simulink model "MotorXploer"  (R2024b)
settings: Solver=FixedStepAuto  StartTime=0.0  StopTime=inf  FixedStep=0.001  RelTol=1e-3  EnableMultiTasking=on
values from neighbouring files (symbols this model uses):
  n = (-(230/0.2)*((Torque1).^2) + 230*Torque1) ./ (((5-0.98)/0.2)*Torque1*12 + 0.98*12)*100    [UnitedPlot.m]
undefined symbols (not defined in the file or in its folder): Blocking, LF, Non
libraries: hdlsllib x5, amg_usbconverter_n_connect_lib x3, cstblocks x1, simulink x1, waijung_addon_module x1
(part 1 of 2)
settings Model: Creator=beamk  LastModifiedBy=KATANA
settings OptimizationCC: DefaultParameterBehavior=Inlined  EnhancedBackFolding=on  PassReuseOutputArgsAs=Individual arguments  ZeroExternalMemoryAtStartup=off  ZeroInternalMemoryAtStartup=off  MaxStackSize=64  OptimizeBlockOrder=speed  DifferentSizesBufferReuse=on  OptimizationCustomize=off  EfficientTunableParamExpr=on
settings DebuggingCC: ParameterTunabilityLossMsg=error
settings HardwareCC: ProdBitPerPointer=32  ProdBitPerSizeT=32  ProdBitPerPtrDiffT=32  ProdLargestAtomicInteger=Long  ProdLargestAtomicFloat=Double  ProdWordSize=32  ProdLongLongMode=on  ProdHWDeviceType=ARM Compatible->ARM Cortex-M
settings SFSimCC: MATLABDynamicMemAlloc=off
settings RTWCC: Description=Embedded Coder  SystemTargetFile=ert.tlc  HardwareBoard=STM32G4xx Based  TemplateMakefile=ert_default_tmf  Toolchain=GNU Tools for ARM Embedded Processors
settings CodeAppCC: ForceParamTrailComments=on  IgnoreCustomStorageClasses=off  OperatorAnnotations=on  SimulinkDataObjDesc=on  SFDataObjDesc=on  InsertBlockDesc=on
settings ERTTargetCC: TargetLangStandard=C99 (ISO)  CodeReplacementLibrary=ARM Cortex-M  ExtModeTransport=3  ExtModeStaticAlloc=on  ExtModeStaticAllocSize=2048  ExtModeMexFile=ext_xcp  ExtModeIntrfLevel=Level2 - Open

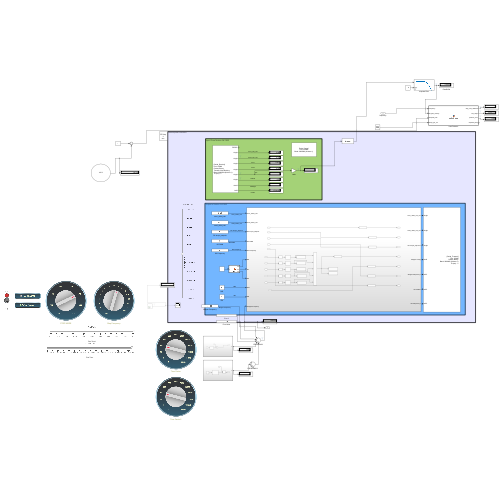
[thumbnail: Simulink's stored preview of the top-level diagram]
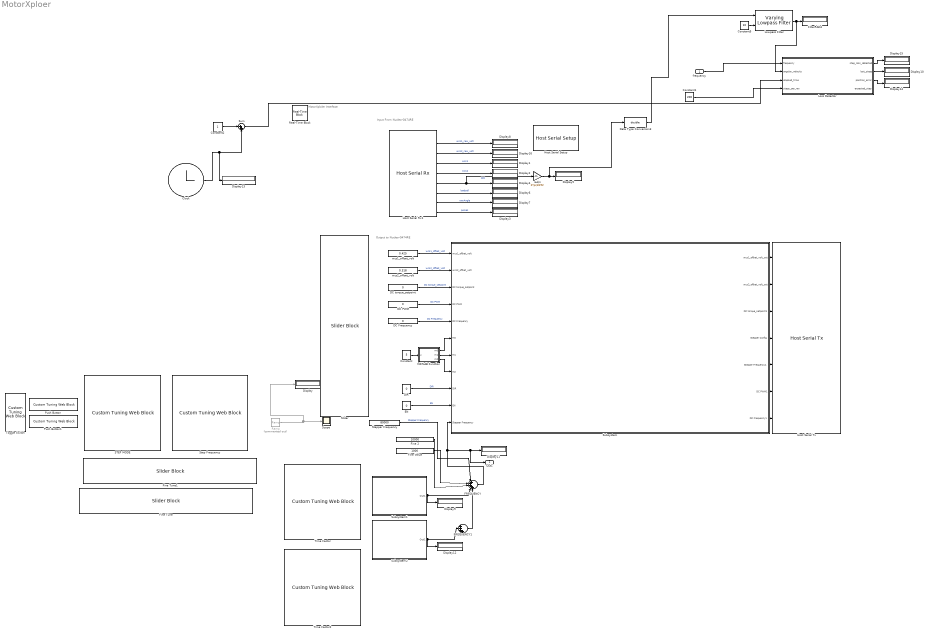
== system MotorXploer ==
  note: Output to Nucleo-G474RE
  note: Input From Nucleo-G474RE
  note: MotorXploler Interface
  frequency : Inport
  Clock : Clock
  Constant : Constant  Value=5
  Constant1 : Constant  Value=200
  Constant2 : Constant
  Constant5 : Constant  Value=10
  DC Frequency : Constant  Value=0
  DC PWM : Constant  Value=0
  DC torque_setpoint : Constant  Value=0
  DIR : Constant  Value=0  OutDataTypeStr=uint8
  Data Type Conversion3 : DataTypeConversion  OutDataTypeStr=double  SaturateOnIntegerOverflow=off  RndMeth=Floor
  Display{,1..16} (17 alike) : Display
  EN : Constant  Value=0  OutDataTypeStr=uint8
  FREQUENCY : Sum  Inputs=|+++++
  FREQUENCY1 : Sum  Inputs=|++++
  FilterRAD4 : Display
  Fine 2 : Constant  Value=10000
  Fine Tune : SliderBlock  ScaleMax=1000
  Fine Tune1 : SliderBlock  ScaleMax=10000  TickInterval=1000
  Fine Value : Constant  Value=1000
  Host Serial Rx1 : amg_usbconverter_n_connect_lib/Host Serial Rx  conf=rx  port=<auto>  baudrate=2000000  databits=8  parity=None  stopbit=1  flowcontrol=None  transfer=Non-Blocking  timeout=5  packetmode=Binary  enableinitialvalues=off  initialvalues=[]  binheader='45'  binterminator='A'  porttype_double=0  porttype_single=6  porttype_int8=0  porttype_uint8=0  porttype_int16=0  porttype_uint16=1  porttype_int32=1  porttype_uint32=0  asciiformat='%f,%f,%d,%d'  rx_asciiterminator="LF (0x0A - \"\\n\")"  tx_asciiterminator="CRLF (0x0D 0x0A - \"\\r\\n\")"  sampletime=-1  enablecustomportlabel=off  cinputportlabel=0  coutputportlabel=A  portpinstr=0  blockid=HostSerialRx1  inputporttype=[]  inputportwidth=[]  inputportlabel={}  outputporttype=[3 1 1 1 1 1 1 5 6]  outputportwidth=[1 1 1 1 1 1 1 1 1]  outputportlabel={'READY','single','single','single','single','single','single','uint16','int32'}  compat=0  optionstring=[]  autoport='COM17'
  Host Serial Setup : amg_usbconverter_n_connect_lib/Host Serial Setup  conf=setup  port=<auto>  baudrate=2000000  databits=8  parity=None  stopbit=1  flowcontrol=None  transfer=Blocking  timeout=2  packetmode=Binary  initialvalues=[]  binheader='7E 7E'  binterminator='03 03'  porttype_double=0  porttype_single=1  porttype_int8=0  porttype_uint8=0  porttype_int16=0  porttype_uint16=0  porttype_int32=0  porttype_uint32=2  asciiformat='%d %u %x'  rx_asciiterminator="CRLF (0x0D 0x0A - \"\\r\\n\")"  tx_asciiterminator="CRLF (0x0D 0x0A - \"\\r\\n\")"  sampletime=-1  enablecustomportlabel=off  cinputportlabel=0  coutputportlabel=A  portpinstr=0  blockid=HostSerialSetup  inputporttype=[]  inputportwidth=[]  inputportlabel={}  outputporttype=[]  outputportwidth=[]  outputportlabel={}  compat=0  optionstring=[]  autoport='COM17'
  Host Serial Tx : amg_usbconverter_n_connect_lib/Host Serial Tx  conf=tx  port=<auto>  baudrate=2000000  databits=8  parity=None  stopbit=1  flowcontrol=None  transfer=Blocking  timeout=2  packetmode=Binary  initialvalues=[]  binheader='45'  binterminator='A'  porttype_double=0  porttype_single=3  porttype_int8=0  porttype_uint8=1  porttype_int16=0  porttype_uint16=0  porttype_int32=3  porttype_uint32=0  asciiformat='%d,%f'  rx_asciiterminator="CRLF (0x0D 0x0A - \"\\r\\n\")"  tx_asciiterminator="CRLF (0x0D 0x0A - \"\\r\\n\")"  sampletime=-1  enablecustomportlabel=off  cinputportlabel=0  coutputportlabel=A  portpinstr=0  blockid=HostSerialTx  inputporttype=[1 1 1 3 6 6 6]  inputportwidth=[1 1 1 1 1 1 1]  inputportlabel={'single','single','single','uint8','int32','int32','int32'}  outputporttype=[]  outputportwidth=[]  outputportlabel={}  compat=0  optionstring=[]  autoport='COM17'
      settings: SourceProductName=aMG USB Converter N
  Loss Detector : MATLAB Function  TreatAsAtomicUnit=on
  Lowpass Filter : cstblocks/Linear Parameter Varying/Varying Lowpass Filter  N=3
  MATLAB Function : MATLAB Function  TreatAsAtomicUnit=on
  Push Button : CustomTuningWebBlock  LabelPosition=Hide  ShowInitialText=on  Configuration="{\"components\":[{\"name\":\"BackgroundImageComponent\",\"settings\":{\"image\":{\"size\":[0,0],\"src\":\"default\",\"srcOrientation\":\"horizontal\"},\"position\":[0,0,1,1],\"scaleMode\":\"0\"}},{\"name\":\"ButtonStateComponent\",\"settings\":{\"buttonType\":\"latch\",\"clickFcn\":\"\",\"image\":{\"size\":[180,45],\"srcOrientation\":\"Right\"},\"latched\":false,\"offValue\":null,\"onValue\":\"1\",\"position\":[0,0,1,1],\"pressDelay\":\"500\",\"pressFcn\":\"\",\"repeatInterval\":\"0\",\"states\":[{\"horizontalAlignment\":\"center\",\"image\":{\"position\":[0.05,0.015,0.98,0.9],\"size\":[0.98,0.9],\"src\":\"data:image\\/svg+xml;base64,PHN2ZyB4bWxucz0iaHR0cDovL3d3dy53My5vcmcvMjAwMC9zdmciIHhtbG5zOnhsaW5rPSJodHRwOi8vd3d3LnczLm9yZy8xOTk5L3hsaW5rIiB2aWV3Qm94PSIwIDAgMTc3LjI1IDQwLjg4Ij48ZGVmcz48c3R5bGU+LmNscy0xe2ZpbGw6dXJsKCNyYWRpYWwtZ3JhZGllbnQpO30uY2xzLTJ7ZmlsbDp1cmwoI2xpbmVhci1ncmFkaWVudCk7fS5jbHMtM3tmaWxsOnVybCgjbGluZWFyLWdyYWRpZW50LTIpO308L3N0eWxlPjxyYWRpYWxHcmFkaWVudCBpZD0icmFkaWFsLWdyYWRpZW50IiBjeD0iOTAuMDkiIGN5PSIyMi42NiIgcj0i ...(+2212 chars)\",\"srcOrientation\":\"Right\"},\"label\":{\"color\":[1,1,0.78,1],\"icon\":{\"size\":[1.2,1.2],\"src\":\"data:image\\/svg+xml;base64,PHN2ZyBpZD0iT2ZmIiB4bWxucz0iaHR0cDovL3d3dy53My5vcmcvMjAwMC9zdmciIHhtbG5zOnhsaW5rPSJodHRwOi8vd3d3LnczLm9yZy8xOTk5L3hsaW5rIiB2aWV3Qm94PSIwIDAgNTAgNTAiPjxkZWZzPjxzdHlsZT4uY2xzLTF7ZmlsbDojN2Y4MDgwO3N0cm9rZTojMjcyNjI2O3N0cm9rZS1taXRlcmxpbWl0OjEwO3N0cm9rZS13aWR0aDozcHg7fS5jbHMtMntmaWxsOnVybCgjbGluZWFyLWdyYWRpZW50KTt9PC9zdHlsZT48bGluZWFyR3JhZGllbnQgaWQ9ImxpbmVhci1ncmFkaWVudCIgeDE9IjI1IiB5MT0iOSIgeDI9IjI1IiB5Mj0iMzciIGdyYWRpZW50VW5pdHM9InVzZXJTcGFjZU9uVXNlIj48c3RvcCBvZmZzZXQ9IjAiIHN0b3AtY29sb3I9IiNmZmYiIHN0b3Atb3BhY2l0eT0iMC43NSIvPjxzdG9wIG9mZnNldD0iMSIgc3RvcC1jb2xvcj0iI2ZmZiIgc3RvcC1vcGFjaXR5PSIwIi8+PC9saW5lYXJHcmFkaWVudD48L2RlZnM+PGNpcmNsZSBjbGFzcz0iY2xzLTEiIGN4PSIyNSIgY3k9IjI1IiByPSIyMCIvPjxjaXJjbGUgY2xhc3M9ImNscy0yIiBjeD0iMjUiIGN5PSIyMyIgcj0iMTQiLz48L3N2Zz4=\",\"srcOrientation\":\"Right\"},\"iconOffset\":0,\"iconPlacement\":\"left\",\"opacity\":1,\"show\":true,\"text\":{\"content\":\"CW_Stepper\",\"font\":\"Helvetica\"}},\"labelOffset\":[-0.025,0],\"verticalAlignment\":\"middle\"},{\"horizontalAlignment\":\"center\",\"image\":{\"position\":[0.05,0.015,0.98,0.9],\"size\":[0.98,0.9],\"src\":\"data:image\\/svg+xml;base64,PHN2ZyB4bWxucz0iaHR0cDovL3d3dy53My5vcmcvMjAwMC9zdmciIHhtbG5zOnhsaW5rPSJodHRwOi8vd3d3LnczLm9yZy8xOTk5L3hsaW5rIiB2aWV3Qm94PSIwIDAgMTc3LjI1IDQwLjg4Ij48ZGVmcz48c3R5bGU+LmNscy0xe2ZpbGw6dXJsKCNyYWRpYWwtZ3JhZGllbnQpO30uY2xzLTJ7ZmlsbDp1cmwoI2xpbmVhci1ncmFkaWVudCk7fS5jbHMtM3tmaWxsOnVybCgjbGluZWFyLWdyYWRpZW50LTIpO308L3N0eWxlPjxyYWRpYWxHcmFkaWVudCBpZD0icmFkaWFsLWdyYWRpZW50IiBjeD0iOTAuMDkiIGN5PSIyMi42NiIgcj0i ...(+2216 chars)\",\"srcOrientation\":\"Right\"},\"label\":{\"color\":[1,1,0.78,1],\"icon\":{\"size\":[1.2,1.2],\"src\":\"data:image\\/svg+xml;base64,PHN2ZyB4bWxucz0iaHR0cDovL3d3dy53My5vcmcvMjAwMC9zdmciIHhtbG5zOnhsaW5rPSJodHRwOi8vd3d3LnczLm9yZy8xOTk5L3hsaW5rIiB2aWV3Qm94PSIwIDAgNTAgNTAiPjxkZWZzPjxzdHlsZT4uY2xzLTF7ZmlsbDojNmFiZDQ1O3N0cm9rZTojMjcyNjI2O3N0cm9rZS1taXRlcmxpbWl0OjEwO3N0cm9rZS13aWR0aDozcHg7fS5jbHMtMntmaWxsOnVybCgjbGluZWFyLWdyYWRpZW50KTt9PC9zdHlsZT48bGluZWFyR3JhZGllbnQgaWQ9ImxpbmVhci1ncmFkaWVudCIgeDE9IjI1IiB5MT0iOSIgeDI9IjI1IiB5Mj0iMzciIGdyYWRpZW50VW5pdHM9InVzZXJTcGFjZU9uVXNlIj48c3RvcCBvZmZzZXQ9IjAiIHN0b3AtY29sb3I9IiNmZmYiIHN0b3Atb3BhY2l0eT0iMC43NSIvPjxzdG9wIG9mZnNldD0iMSIgc3RvcC1jb2xvcj0iI2ZmZiIgc3RvcC1vcGFjaXR5PSIwIi8+PC9saW5lYXJHcmFkaWVudD48L2RlZnM+PGcgaWQ9Ik9uIj48Y2lyY2xlIGNsYXNzPSJjbHMtMSIgY3g9IjI1IiBjeT0iMjUiIHI9IjIwIi8+PGNpcmNsZSBjbGFzcz0iY2xzLTIiIGN4PSIyNSIgY3k9IjIzIiByPSIxNCIvPjwvZz48L3N2Zz4=\",\"srcOrientation\":\"Right\"},\"iconOffset\":0,\"iconPlacement\":\"left\",\"opacity\":1,\"show\":true,\"text\":{\"content\":\"CW_Stepper\",\"font\":\"Helvetica\"}},\"labelOffset\":[0,0],\"verticalAlignment\":\"middle\"},{\"horizontalAlignment\":\"center\",\"image\":{\"position\":[0.05,0.015,0.98,0.9],\"size\":[0.98,0.9],\"src\":\"data:image\\/svg+xml;base64,PHN2ZyB4bWxucz0iaHR0cDovL3d3dy53My5vcmcvMjAwMC9zdmciIHhtbG5zOnhsaW5rPSJodHRwOi8vd3d3LnczLm9yZy8xOTk5L3hsaW5rIiB2aWV3Qm94PSIwIDAgMTc3LjI1IDQwLjg4Ij48ZGVmcz48c3R5bGU+LmNscy0xe2ZpbGw6dXJsKCNyYWRpYWwtZ3JhZGllbnQpO30uY2xzLTJ7ZmlsbDp1cmwoI2xpbmVhci1ncmFkaWVudCk7fS5jbHMtM3tmaWxsOnVybCgjbGluZWFyLWdyYWRpZW50LTIpO308L3N0eWxlPjxyYWRpYWxHcmFkaWVudCBpZD0icmFkaWFsLWdyYWRpZW50IiBjeD0iOTAuMDkiIGN5PSIyMi42NiIgcj0i ...(+2212 chars)\",\"srcOrientation\":\"Right\"},\"label\":{\"color\":[1,1,0.78,1],\"icon\":{\"size\":[1.2,1.2],\"src\":\"data:image\\/svg+xml;base64,PHN2ZyB4bWxucz0iaHR0cDovL3d3dy53My5vcmcvMjAwMC9zdmciIHhtbG5zOnhsaW5rPSJodHRwOi8vd3d3LnczLm9yZy8xOTk5L3hsaW5rIiB2aWV3Qm94PSIwIDAgNTAgNTAiPjxkZWZzPjxzdHlsZT4uY2xzLTF7ZmlsbDojNmFiZDQ1O3N0cm9rZTojMjcyNjI2O3N0cm9rZS1taXRlcmxpbWl0OjEwO3N0cm9rZS13aWR0aDozcHg7fS5jbHMtMntmaWxsOnVybCgjbGluZWFyLWdyYWRpZW50KTt9PC9zdHlsZT48bGluZWFyR3JhZGllbnQgaWQ9ImxpbmVhci1ncmFkaWVudCIgeDE9IjI1IiB5MT0iOSIgeDI9IjI1IiB5Mj0iMzciIGdyYWRpZW50VW5pdHM9InVzZXJTcGFjZU9uVXNlIj48c3RvcCBvZmZzZXQ9IjAiIHN0b3AtY29sb3I9IiNmZmYiIHN0b3Atb3BhY2l0eT0iMC43NSIvPjxzdG9wIG9mZnNldD0iMSIgc3RvcC1jb2xvcj0iI2ZmZiIgc3RvcC1vcGFjaXR5PSIwIi8+PC9saW5lYXJHcmFkaWVudD48L2RlZnM+PGcgaWQ9Ik9uIj48Y2lyY2xlIGNsYXNzPSJjbHMtMSIgY3g9IjI1IiBjeT0iMjUiIHI9IjIwIi8+PGNpcmNsZSBjbGFzcz0iY2xzLTIiIGN4PSIyNSIgY3k9IjIzIiByPSIxNCIvPjwvZz48L3N2Zz4=\",\"srcOrientation\":\"Right\"},\"iconOffset\":0,\"iconPlacement\":\"left\",\"opacity\":1,\"show\":true,\"text\":{\"content\":\"CW_Stepper\",\"font\":\"Helvetica\"}},\"labelOffset\":[-0.025,0],\"verticalAlignment\":\"middle\"},{\"horizontalAlignment\":\"center\",\"image\":{\"position\":[0.05,0.015,0.98,0.9],\"size\":[0.98,0.9],\"src\":\"data:image\\/svg+xml;base64,PHN2ZyB4bWxucz0iaHR0cDovL3d3dy53My5vcmcvMjAwMC9zdmciIHhtbG5zOnhsaW5rPSJodHRwOi8vd3d3LnczLm9yZy8xOTk5L3hsaW5rIiB2aWV3Qm94PSIwIDAgMTc3LjI1IDQwLjg4Ij48ZGVmcz48c3R5bGU+LmNscy0xe2ZpbGw6dXJsKCNyYWRpYWwtZ3JhZGllbnQpO30uY2xzLTJ7ZmlsbDp1cmwoI2xpbmVhci1ncmFkaWVudCk7fS5jbHMtM3tmaWxsOnVybCgjbGluZWFyLWdyYWRpZW50LTIpO308L3N0eWxlPjxyYWRpYWxHcmFkaWVudCBpZD0icmFkaWFsLWdyYWRpZW50IiBjeD0iOTAuMDkiIGN5PSIyMi42NiIgcj0i ...(+2216 chars)\",\"srcOrientation\":\"Right\"},\"label\":{\"color\":[1,1,0.78,1],\"icon\":{\"size\":[1.2,1.2],\"src\":\"data:image\\/svg+xml;base64,PHN2ZyBpZD0iT2ZmIiB4bWxucz0iaHR0cDovL3d3dy53My5vcmcvMjAwMC9zdmciIHhtbG5zOnhsaW5rPSJodHRwOi8vd3d3LnczLm9yZy8xOTk5L3hsaW5rIiB2aWV3Qm94PSIwIDAgNTAgNTAiPjxkZWZzPjxzdHlsZT4uY2xzLTF7ZmlsbDojN2Y4MDgwO3N0cm9rZTojMjcyNjI2O3N0cm9rZS1taXRlcmxpbWl0OjEwO3N0cm9rZS13aWR0aDozcHg7fS5jbHMtMntmaWxsOnVybCgjbGluZWFyLWdyYWRpZW50KTt9PC9zdHlsZT48bGluZWFyR3JhZGllbnQgaWQ9ImxpbmVhci1ncmFkaWVudCIgeDE9IjI1IiB5MT0iOSIgeDI9IjI1IiB5Mj0iMzciIGdyYWRpZW50VW5pdHM9InVzZXJTcGFjZU9uVXNlIj48c3RvcCBvZmZzZXQ9IjAiIHN0b3AtY29sb3I9IiNmZmYiIHN0b3Atb3BhY2l0eT0iMC43NSIvPjxzdG9wIG9mZnNldD0iMSIgc3RvcC1jb2xvcj0iI2ZmZiIgc3RvcC1vcGFjaXR5PSIwIi8+PC9saW5lYXJHcmFkaWVudD48L2RlZnM+PGNpcmNsZSBjbGFzcz0iY2xzLTEiIGN4PSIyNSIgY3k9IjI1IiByPSIyMCIvPjxjaXJjbGUgY2xhc3M9ImNscy0yIiBjeD0iMjUiIGN5PSIyMyIgcj0iMTQiLz48L3N2Zz4=\",\"srcOrientation\":\"Right\"},\"iconOffset\":0,\"iconPlacement\":\"left\",\"opacity\":1,\"show\":true,\"text\":{\"content\":\"CW_Stepper\",\"font\":\"Helvetica\"}},\"labelOffset\":[0,0],\"verticalAlignment\":\"middle\"}]}},{\"name\":\"ForegroundImageComponent\",\"settings\":{\"image\":{\"size\":[0,0],\"src\":\"default\",\"srcOrientation\":\"horizontal\"},\"isForeground\":1,\"position\":[0,0,1,1],\"scaleMode\":\"0\"}}],\"settings\":{\"BindingType\":\"param\",\"aspectRatio\":3.7777777777777777,\"backgroundColor\":[0,0,0,\"1\"],\"backgroundOffset\":0,\"backgroundOpacity\":1,\"fixedAspectRatio\":\"on\",\"foregroundColor\":[252,252,196],\"showBackgroundColor\":false,\"variant\":\"push\",\"version\":\"R2024b\"},\"type\":\"Button\"}"
  Push Button1 : CustomTuningWebBlock  LabelPosition=Hide  ShowInitialText=on  Configuration="{\"components\":[{\"name\":\"BackgroundImageComponent\",\"settings\":{\"image\":{\"size\":[0,0],\"src\":\"default\",\"srcOrientation\":\"horizontal\"},\"position\":[0,0,1,1],\"scaleMode\":\"0\"}},{\"name\":\"ButtonStateComponent\",\"settings\":{\"buttonType\":\"latch\",\"clickFcn\":\"\",\"image\":{\"size\":[180,45],\"srcOrientation\":\"Right\"},\"latched\":true,\"offValue\":1,\"onValue\":\"0\",\"position\":[0,0,1,1],\"pressDelay\":\"500\",\"pressFcn\":\"\",\"repeatInterval\":\"0\",\"states\":[{\"horizontalAlignment\":\"center\",\"image\":{\"position\":[0.05,0.015,0.98,0.9],\"size\":[0.98,0.9],\"src\":\"data:image\\/svg+xml;base64,PHN2ZyB4bWxucz0iaHR0cDovL3d3dy53My5vcmcvMjAwMC9zdmciIHhtbG5zOnhsaW5rPSJodHRwOi8vd3d3LnczLm9yZy8xOTk5L3hsaW5rIiB2aWV3Qm94PSIwIDAgMTc3LjI1IDQwLjg4Ij48ZGVmcz48c3R5bGU+LmNscy0xe2ZpbGw6dXJsKCNyYWRpYWwtZ3JhZGllbnQpO30uY2xzLTJ7ZmlsbDp1cmwoI2xpbmVhci1ncmFkaWVudCk7fS5jbHMtM3tmaWxsOnVybCgjbGluZWFyLWdyYWRpZW50LTIpO308L3N0eWxlPjxyYWRpYWxHcmFkaWVudCBpZD0icmFkaWFsLWdyYWRpZW50IiBjeD0iOTAuMDkiIGN5PSIyMi42NiIgcj0i ...(+2212 chars)\",\"srcOrientation\":\"Right\"},\"label\":{\"color\":[1,1,0.78,1],\"icon\":{\"size\":[1.2,1.2],\"src\":\"data:image\\/svg+xml;base64,PHN2ZyBpZD0iT2ZmIiB4bWxucz0iaHR0cDovL3d3dy53My5vcmcvMjAwMC9zdmciIHhtbG5zOnhsaW5rPSJodHRwOi8vd3d3LnczLm9yZy8xOTk5L3hsaW5rIiB2aWV3Qm94PSIwIDAgNTAgNTAiPjxkZWZzPjxzdHlsZT4uY2xzLTF7ZmlsbDojN2Y4MDgwO3N0cm9rZTojMjcyNjI2O3N0cm9rZS1taXRlcmxpbWl0OjEwO3N0cm9rZS13aWR0aDozcHg7fS5jbHMtMntmaWxsOnVybCgjbGluZWFyLWdyYWRpZW50KTt9PC9zdHlsZT48bGluZWFyR3JhZGllbnQgaWQ9ImxpbmVhci1ncmFkaWVudCIgeDE9IjI1IiB5MT0iOSIgeDI9IjI1IiB5Mj0iMzciIGdyYWRpZW50VW5pdHM9InVzZXJTcGFjZU9uVXNlIj48c3RvcCBvZmZzZXQ9IjAiIHN0b3AtY29sb3I9IiNmZmYiIHN0b3Atb3BhY2l0eT0iMC43NSIvPjxzdG9wIG9mZnNldD0iMSIgc3RvcC1jb2xvcj0iI2ZmZiIgc3RvcC1vcGFjaXR5PSIwIi8+PC9saW5lYXJHcmFkaWVudD48L2RlZnM+PGNpcmNsZSBjbGFzcz0iY2xzLTEiIGN4PSIyNSIgY3k9IjI1IiByPSIyMCIvPjxjaXJjbGUgY2xhc3M9ImNscy0yIiBjeD0iMjUiIGN5PSIyMyIgcj0iMTQiLz48L3N2Zz4=\",\"srcOrientation\":\"Right\"},\"iconOffset\":0,\"iconPlacement\":\"left\",\"opacity\":1,\"show\":true,\"text\":{\"content\":\"CCW_Stepper \",\"font\":\"Helvetica\"}},\"labelOffset\":[-0.025,0],\"verticalAlignment\":\"middle\"},{\"horizontalAlignment\":\"center\",\"image\":{\"position\":[0.05,0.015,0.98,0.9],\"size\":[0.98,0.9],\"src\":\"data:image\\/svg+xml;base64,PHN2ZyB4bWxucz0iaHR0cDovL3d3dy53My5vcmcvMjAwMC9zdmciIHhtbG5zOnhsaW5rPSJodHRwOi8vd3d3LnczLm9yZy8xOTk5L3hsaW5rIiB2aWV3Qm94PSIwIDAgMTc3LjI1IDQwLjg4Ij48ZGVmcz48c3R5bGU+LmNscy0xe2ZpbGw6dXJsKCNyYWRpYWwtZ3JhZGllbnQpO30uY2xzLTJ7ZmlsbDp1cmwoI2xpbmVhci1ncmFkaWVudCk7fS5jbHMtM3tmaWxsOnVybCgjbGluZWFyLWdyYWRpZW50LTIpO308L3N0eWxlPjxyYWRpYWxHcmFkaWVudCBpZD0icmFkaWFsLWdyYWRpZW50IiBjeD0iOTAuMDkiIGN5PSIyMi42NiIgcj0i ...(+2216 chars)\",\"srcOrientation\":\"Right\"},\"label\":{\"color\":[1,1,0.78,1],\"icon\":{\"size\":[1.2,1.2],\"src\":\"data:image\\/svg+xml;base64,PHN2ZyB4bWxucz0iaHR0cDovL3d3dy53My5vcmcvMjAwMC9zdmciIHhtbG5zOnhsaW5rPSJodHRwOi8vd3d3LnczLm9yZy8xOTk5L3hsaW5rIiB2aWV3Qm94PSIwIDAgNTAgNTAiPjxkZWZzPjxzdHlsZT4uY2xzLTF7ZmlsbDojNmFiZDQ1O3N0cm9rZTojMjcyNjI2O3N0cm9rZS1taXRlcmxpbWl0OjEwO3N0cm9rZS13aWR0aDozcHg7fS5jbHMtMntmaWxsOnVybCgjbGluZWFyLWdyYWRpZW50KTt9PC9zdHlsZT48bGluZWFyR3JhZGllbnQgaWQ9ImxpbmVhci1ncmFkaWVudCIgeDE9IjI1IiB5MT0iOSIgeDI9IjI1IiB5Mj0iMzciIGdyYWRpZW50VW5pdHM9InVzZXJTcGFjZU9uVXNlIj48c3RvcCBvZmZzZXQ9IjAiIHN0b3AtY29sb3I9IiNmZmYiIHN0b3Atb3BhY2l0eT0iMC43NSIvPjxzdG9wIG9mZnNldD0iMSIgc3RvcC1jb2xvcj0iI2ZmZiIgc3RvcC1vcGFjaXR5PSIwIi8+PC9saW5lYXJHcmFkaWVudD48L2RlZnM+PGcgaWQ9Ik9uIj48Y2lyY2xlIGNsYXNzPSJjbHMtMSIgY3g9IjI1IiBjeT0iMjUiIHI9IjIwIi8+PGNpcmNsZSBjbGFzcz0iY2xzLTIiIGN4PSIyNSIgY3k9IjIzIiByPSIxNCIvPjwvZz48L3N2Zz4=\",\"srcOrientation\":\"Right\"},\"iconOffset\":0,\"iconPlacement\":\"left\",\"opacity\":1,\"show\":true,\"text\":{\"content\":\"CCW_Stepper \",\"font\":\"Helvetica\"}},\"labelOffset\":[0,0],\"verticalAlignment\":\"middle\"},{\"horizontalAlignment\":\"center\",\"image\":{\"position\":[0.05,0.015,0.98,0.9],\"size\":[0.98,0.9],\"src\":\"data:image\\/svg+xml;base64,PHN2ZyB4bWxucz0iaHR0cDovL3d3dy53My5vcmcvMjAwMC9zdmciIHhtbG5zOnhsaW5rPSJodHRwOi8vd3d3LnczLm9yZy8xOTk5L3hsaW5rIiB2aWV3Qm94PSIwIDAgMTc3LjI1IDQwLjg4Ij48ZGVmcz48c3R5bGU+LmNscy0xe2ZpbGw6dXJsKCNyYWRpYWwtZ3JhZGllbnQpO30uY2xzLTJ7ZmlsbDp1cmwoI2xpbmVhci1ncmFkaWVudCk7fS5jbHMtM3tmaWxsOnVybCgjbGluZWFyLWdyYWRpZW50LTIpO308L3N0eWxlPjxyYWRpYWxHcmFkaWVudCBpZD0icmFkaWFsLWdyYWRpZW50IiBjeD0iOTAuMDkiIGN5PSIyMi42NiIgcj0i ...(+2212 chars)\",\"srcOrientation\":\"Right\"},\"label\":{\"color\":[1,1,0.78,1],\"icon\":{\"size\":[1.2,1.2],\"src\":\"data:image\\/svg+xml;base64,PHN2ZyB4bWxucz0iaHR0cDovL3d3dy53My5vcmcvMjAwMC9zdmciIHhtbG5zOnhsaW5rPSJodHRwOi8vd3d3LnczLm9yZy8xOTk5L3hsaW5rIiB2aWV3Qm94PSIwIDAgNTAgNTAiPjxkZWZzPjxzdHlsZT4uY2xzLTF7ZmlsbDojNmFiZDQ1O3N0cm9rZTojMjcyNjI2O3N0cm9rZS1taXRlcmxpbWl0OjEwO3N0cm9rZS13aWR0aDozcHg7fS5jbHMtMntmaWxsOnVybCgjbGluZWFyLWdyYWRpZW50KTt9PC9zdHlsZT48bGluZWFyR3JhZGllbnQgaWQ9ImxpbmVhci1ncmFkaWVudCIgeDE9IjI1IiB5MT0iOSIgeDI9IjI1IiB5Mj0iMzciIGdyYWRpZW50VW5pdHM9InVzZXJTcGFjZU9uVXNlIj48c3RvcCBvZmZzZXQ9IjAiIHN0b3AtY29sb3I9IiNmZmYiIHN0b3Atb3BhY2l0eT0iMC43NSIvPjxzdG9wIG9mZnNldD0iMSIgc3RvcC1jb2xvcj0iI2ZmZiIgc3RvcC1vcGFjaXR5PSIwIi8+PC9saW5lYXJHcmFkaWVudD48L2RlZnM+PGcgaWQ9Ik9uIj48Y2lyY2xlIGNsYXNzPSJjbHMtMSIgY3g9IjI1IiBjeT0iMjUiIHI9IjIwIi8+PGNpcmNsZSBjbGFzcz0iY2xzLTIiIGN4PSIyNSIgY3k9IjIzIiByPSIxNCIvPjwvZz48L3N2Zz4=\",\"srcOrientation\":\"Right\"},\"iconOffset\":0,\"iconPlacement\":\"left\",\"opacity\":1,\"show\":true,\"text\":{\"content\":\"CCW_Stepper \",\"font\":\"Helvetica\"}},\"labelOffset\":[-0.025,0],\"verticalAlignment\":\"middle\"},{\"horizontalAlignment\":\"center\",\"image\":{\"position\":[0.05,0.015,0.98,0.9],\"size\":[0.98,0.9],\"src\":\"data:image\\/svg+xml;base64,PHN2ZyB4bWxucz0iaHR0cDovL3d3dy53My5vcmcvMjAwMC9zdmciIHhtbG5zOnhsaW5rPSJodHRwOi8vd3d3LnczLm9yZy8xOTk5L3hsaW5rIiB2aWV3Qm94PSIwIDAgMTc3LjI1IDQwLjg4Ij48ZGVmcz48c3R5bGU+LmNscy0xe2ZpbGw6dXJsKCNyYWRpYWwtZ3JhZGllbnQpO30uY2xzLTJ7ZmlsbDp1cmwoI2xpbmVhci1ncmFkaWVudCk7fS5jbHMtM3tmaWxsOnVybCgjbGluZWFyLWdyYWRpZW50LTIpO308L3N0eWxlPjxyYWRpYWxHcmFkaWVudCBpZD0icmFkaWFsLWdyYWRpZW50IiBjeD0iOTAuMDkiIGN5PSIyMi42NiIgcj0i ...(+2216 chars)\",\"srcOrientation\":\"Right\"},\"label\":{\"color\":[1,1,0.78,1],\"icon\":{\"size\":[1.2,1.2],\"src\":\"data:image\\/svg+xml;base64,PHN2ZyBpZD0iT2ZmIiB4bWxucz0iaHR0cDovL3d3dy53My5vcmcvMjAwMC9zdmciIHhtbG5zOnhsaW5rPSJodHRwOi8vd3d3LnczLm9yZy8xOTk5L3hsaW5rIiB2aWV3Qm94PSIwIDAgNTAgNTAiPjxkZWZzPjxzdHlsZT4uY2xzLTF7ZmlsbDojN2Y4MDgwO3N0cm9rZTojMjcyNjI2O3N0cm9rZS1taXRlcmxpbWl0OjEwO3N0cm9rZS13aWR0aDozcHg7fS5jbHMtMntmaWxsOnVybCgjbGluZWFyLWdyYWRpZW50KTt9PC9zdHlsZT48bGluZWFyR3JhZGllbnQgaWQ9ImxpbmVhci1ncmFkaWVudCIgeDE9IjI1IiB5MT0iOSIgeDI9IjI1IiB5Mj0iMzciIGdyYWRpZW50VW5pdHM9InVzZXJTcGFjZU9uVXNlIj48c3RvcCBvZmZzZXQ9IjAiIHN0b3AtY29sb3I9IiNmZmYiIHN0b3Atb3BhY2l0eT0iMC43NSIvPjxzdG9wIG9mZnNldD0iMSIgc3RvcC1jb2xvcj0iI2ZmZiIgc3RvcC1vcGFjaXR5PSIwIi8+PC9saW5lYXJHcmFkaWVudD48L2RlZnM+PGNpcmNsZSBjbGFzcz0iY2xzLTEiIGN4PSIyNSIgY3k9IjI1IiByPSIyMCIvPjxjaXJjbGUgY2xhc3M9ImNscy0yIiBjeD0iMjUiIGN5PSIyMyIgcj0iMTQiLz48L3N2Zz4=\",\"srcOrientation\":\"Right\"},\"iconOffset\":0,\"iconPlacement\":\"left\",\"opacity\":1,\"show\":true,\"text\":{\"content\":\"CCW_Stepper \",\"font\":\"Helvetica\"}},\"labelOffset\":[0,0],\"verticalAlignment\":\"middle\"}]}},{\"name\":\"ForegroundImageComponent\",\"settings\":{\"image\":{\"size\":[0,0],\"src\":\"default\",\"srcOrientation\":\"horizontal\"},\"isForeground\":1,\"position\":[0,0,1,1],\"scaleMode\":\"0\"}}],\"settings\":{\"BindingType\":\"param\",\"aspectRatio\":3.7777777777777777,\"backgroundColor\":[0,0,0,\"1\"],\"backgroundOffset\":0,\"backgroundOpacity\":1,\"fixedAspectRatio\":\"on\",\"foregroundColor\":[252,252,196],\"showBackgroundColor\":false,\"variant\":\"push\",\"version\":\"R2024b\"},\"type\":\"Button\"}"
  Ramp : simulink/Sources/Ramp  Commented=on  slope=1.22  start=0  InitialOutput=0
  Real-Time Block : waijung_addon_module/Real-Time Block  Priority=0  setting=Default  sampletime=-1
      settings: SourceProductName=Misc
  STEP MODE : CustomTuningWebBlock  LabelPosition=Hide  ShowInitialText=on  Configuration="{\"components\":[{\"name\":\"RotarySwitchComponent\",\"settings\":{\"arcAngle\":300,\"arcAngleOffset\":120,\"handle\":{\"size\":[150,150],\"src\":\"data:image\\/svg+xml;base64,PHN2ZyBpZD0iTGF5ZXJfMSIgZGF0YS1uYW1lPSJMYXllciAxIiB4bWxucz0iaHR0cDovL3d3dy53My5vcmcvMjAwMC9zdmciIHhtbG5zOnhsaW5rPSJodHRwOi8vd3d3LnczLm9yZy8xOTk5L3hsaW5rIiB2aWV3Qm94PSIwIDAgMTIxIDEyMSI+PGRlZnM+PHN0eWxlPi5jbHMtMXtmaWxsOnVybCgjbGluZWFyLWdyYWRpZW50KTt9LmNscy0yLC5jbHMtM3tmaWxsOiNkMWQxZDE7fS5jbHMtM3tzdHJva2U6I2I3YjdiNztzdHJva2UtbWl0ZXJsaW1pdDoxMDtzdHJva2Utd2lkdGg6MC4yNXB4O30uY2xzLTR7ZmlsbDojZjMwMDAwO30uY2xzLTV7ZmlsbDojZjIxNzY3O308L3N0eWxlPjxsaW5lYXJHcmFkaWVudCBpZD0ibGluZWFyLWdyYWRpZW50IiB4MT0iNjAuNSIgeTE9IjEyMC41IiB4Mj0iNjAuNSIgeTI9IjAuNSIgZ3JhZGllbnRVbml0cz0idXNlclNwYWNlT25Vc2UiPjxzdG9wIG9mZnNldD0iMCIgc3RvcC1jb2xvcj0iI2QxZDFkMSIvPjxzdG9wIG9mZnNldD0iMC4xIiBzdG9wLWNvbG9yPSIjY2VjZWNlIi8+PHN0b3Agb2Zmc2V0PSIwLjE5IiBzdG9wLWNvbG9yPSIjYzNjM2MzIi8+PHN0b3Agb2Zmc2V0PSIwLjI4IiBzdG9wLWNvbG9yPSIjYjFiMWIxIi8+PHN0b3Agb2Zmc2V0PSIwLjM2IiBzdG9wLWNvbG9yPSIjOTg5ODk4Ii8+PHN0b3Agb2Zmc2V0PSIwLjQ0IiBzdG9wLWNvbG9yPSIjNzg3ODc4Ii8+PHN0b3Agb2Zmc2V0PSIwLjQ2IiBzdG9wLWNvbG9yPSIjNmI2YjZiIi8+PHN0b3Agb2Zmc2V0PSIwLjU0IiBzdG9wLWNvbG9yPSIjNmI2YjZiIi8+PHN0b3Agb2Zmc2V0PSIwLjU2IiBzdG9wLWNvbG9yPSIjNzY3Njc2Ii8+PHN0b3Agb2Zmc2V0PSIwLjY0IiBzdG9wLWNvbG9yPSIjOTc5Nzk3Ii8+PHN0b3Agb2Zmc2V0PSIwLjcyIiBzdG9wLWNvbG9yPSIjYjBiMGIwIi8+PHN0b3Agb2Zmc2V0PSIwLjgxIiBzdG9wLWNvbG9yPSIjYzNjM2MzIi8+PHN0b3Agb2Zmc2V0PSIwLjkiIHN0b3AtY29sb3I9IiNjZGNkY2QiLz48c3RvcCBvZmZzZXQ9IjEiIHN0b3AtY29sb3I9IiNkMWQxZDEiLz48L2xpbmVhckdyYWRpZW50PjwvZGVmcz48Y2lyY2xlIGNsYXNzPSJjbHMtMSIgY3g9IjYwLjUiIGN5PSI2MC41IiByPSI2MCIvPjxwYXRoIGNsYXNzPSJjbHMtMiIgZD0iTTYwLjUsMUE1OS41LDU5LjUsMCwxLDEsMSw2MC41LDU5LjU3LDU5LjU3LDAsMCwxLDYwLjUsMW0wLTFBNjAuNSw2MC41LDAsMSwwLDEyMSw2MC41LDYwLjUsNjAuNSwwLDAsMCw2MC41LDBaIi8+PHJlY3QgY2xhc3M9ImNscy0zIiB4PSIwLjUiIHk9IjUxLjUiIHdpZHRoPSIxMjAiIGhlaWdodD0iMTgiIHJ4PSIzLjA0Ii8+PHJlY3QgY2xhc3M9ImNscy00IiB4PSI1Ljc1IiB5PSI1OC43NSIgd2lkdGg9IjE2IiBoZWlnaHQ9IjMiLz48cGF0aCBjbGFzcz0iY2xzLTUiIGQ9Ik0yMS4yNSw1OS4yNXYyaC0xNXYtMmgxNW0xLTFoLTE3djRoMTd2LTRaIi8+PC9zdmc+\"},\"handleOffset\":[0,0],\"handleOrientation\":180,\"handlePosition\":[0,0,1,1],\"handleSize\":{\"height\":0.5,\"width\":0.5},\"labelRadius\":0.36,\"position\":[0,0,1,1],\"states\":[{\"Label\":{\"color\":[0,0,0,1],\"icon\":{\"size\":[0,0],\"src\":[],\"srcOrientation\":\"Right\"},\"iconOffset\":0,\"iconPlacement\":\"left\",\"opacity\":1,\"position\":[0.7345552884615385,0.6796274038461538],\"show\":true,\"text\":{\"content\":\"Full\",\"font\":\"Helvetica\"}},\"Value\":0},{\"Label\":{\"color\":[0,0,0,1],\"icon\":{\"size\":[0,0],\"src\":[],\"srcOrientation\":\"Right\"},\"iconOffset\":0,\"iconPlacement\":\"left\",\"opacity\":1,\"position\":[0.7191706730769231,0.19501201923076922],\"show\":true,\"text\":{\"content\":\"1\\/2\",\"font\":\"Helvetica\"}},\"Value\":1},{\"Label\":{\"color\":[0,0,0,1],\"icon\":{\"size\":[0,0],\"src\":[],\"srcOrientation\":\"Right\"},\"iconOffset\":0,\"iconPlacement\":\"left\",\"opacity\":1,\"position\":[0.7191706730769231,0.19501201923076922],\"show\":true,\"text\":{\"content\":\"1\\/4\",\"font\":\"Helvetica\"}},\"Value\":2},{\"Label\":{\"color\":[0,0,0,1],\"icon\":{\"size\":[0,0],\"src\":[],\"srcOrientation\":\"Right\"},\"iconOffset\":0,\"iconPlacement\":\"left\",\"opacity\":1,\"position\":[0.7191706730769231,0.19501201923076922],\"show\":true,\"text\":{\"content\":\"1\\/8\",\"font\":\"Helvetica\"}},\"Value\":3},{\"Label\":{\"color\":[0,0,0,1],\"icon\":{\"size\":[0,0],\"src\":[],\"srcOrientation\":\"Right\"},\"iconOffset\":0,\"iconPlacement\":\"left\",\"opacity\":1,\"position\":[0.7191706730769231,0.19501201923076922],\"show\":true,\"text\":{\"content\":\"1\\/16\",\"font\":\"Helvetica\"}},\"Value\":4},{\"Label\":{\"color\":[0,0,0,1],\"icon\":{\"size\":[0,0],\"src\":[],\"srcOrientation\":\"Right\"},\"iconOffset\":0,\"iconPlacement\":\"left\",\"opacity\":1,\"position\":[0.7191706730769231,0.19501201923076922],\"show\":true,\"text\":{\"content\":\"1\\/32\",\"font\":\"Helvetica\"}},\"Value\":5},{\"Label\":{\"color\":[0,0,0,1],\"icon\":{\"size\":[0,0],\"src\":[],\"srcOrientation\":\"Right\"},\"iconOffset\":0,\"iconPlacement\":\"left\",\"opacity\":1,\"position\":[0.7191706730769231,0.19501201923076922],\"show\":true,\"text\":{\"content\":\"1\\/32\",\"font\":\"Helvetica\"}},\"Value\":6},{\"Label\":{\"color\":[0,0,0,1],\"icon\":{\"size\":[0,0],\"src\":[],\"srcOrientation\":\"Right\"},\"iconOffset\":0,\"iconPlacement\":\"left\",\"opacity\":1,\"position\":[0.7191706730769231,0.19501201923076922],\"show\":true,\"text\":{\"content\":\"1\\/32\",\"font\":\"Helvetica\"}},\"Value\":7}],\"tickRadius\":0.32}},{\"name\":\"BackgroundImageComponent\",\"settings\":{\"image\":{\"size\":[155,150],\"src\":\"data:image\\/svg+xml;base64,PD94bWwgdmVyc2lvbj0iMS4wIiBlbmNvZGluZz0idXRmLTgiPz4NCjwhLS0gR2VuZXJhdG9yOiBBZG9iZSBJbGx1c3RyYXRvciAyNS4wLjAsIFNWRyBFeHBvcnQgUGx1Zy1JbiAuIFNWRyBWZXJzaW9uOiA2LjAwIEJ1aWxkIDApICAtLT4NCjxzdmcgdmVyc2lvbj0iMS4xIg0KCSBpZD0iTGF5ZXJfMl8xXyIgeG1sbnM6Y2M9Imh0dHA6Ly9jcmVhdGl2ZWNvbW1vbnMub3JnL25zIyIgeG1sbnM6ZGM9Imh0dHA6Ly9wdXJsLm9yZy9kYy9lbGVtZW50cy8xLjEvIiB4bWxuczppbmtzY2FwZT0iaHR0cDovL3d3dy5pbmtzY2FwZS5vcmcv ...(+4184 chars)\",\"srcOrientation\":\"Right\"},\"position\":[0,0,1,1],\"scaleMode\":\"0\"}},{\"name\":\"ForegroundImageComponent\",\"settings\":{\"image\":{\"size\":[0,0],\"src\":\"default\",\"srcOrientation\":[]},\"isForeground\":1,\"position\":[0,0,1,1],\"scaleMode\":\"0\"}}],\"settings\":{\"BindingType\":\"param\",\"backgroundColor\":[0,0,255,\"1\"],\"backgroundOffset\":1,\"fixedAspectRatio\":\"on\",\"image\":{\"size\":[150,150],\"src\":\"data:image\\/svg+xml;base64,PD94bWwgdmVyc2lvbj0iMS4wIiBlbmNvZGluZz0iVVRGLTgiIHN0YW5kYWxvbmU9Im5vIj8+CjwhLS0gR2VuZXJhdG9yOiBBZG9iZSBJbGx1c3RyYXRvciAxOS4yLjEsIFNWRyBFeHBvcnQgUGx1Zy1JbiAuIFNWRyBWZXJzaW9uOiA2LjAwIEJ1aWxkIDApICAtLT4KCjxzdmcKICAgeG1sbnM6ZGM9Imh0dHA6Ly9wdXJsLm9yZy9kYy9lbGVtZW50cy8xLjEvIgogICB4bWxuczpjYz0iaHR0cDovL2NyZWF0aXZlY29tbW9ucy5vcmcvbnMjIgogICB4bWxuczpyZGY9Imh0dHA6Ly93d3cudzMub3JnLzE5OTkvMDIvMjItcmRmLXN5bnRh ...(+9660 chars)\"},\"showBackgroundColor\":false,\"variant\":\"rotarySwitch\",\"version\":\"R2023a\"},\"type\":\"RotarySwitch\"}"
  Scope : Scope
  Slider : SliderBlock  ScaleMin=-65535  ScaleMax=65535
  Step Frequency : CustomTuningWebBlock  LabelPosition=Hide  ShowInitialText=on  Configuration="{\"components\":[{\"name\":\"RotarySwitchComponent\",\"settings\":{\"arcAngle\":300,\"arcAngleOffset\":120,\"handle\":{\"size\":[150,150],\"src\":\"data:image\\/svg+xml;base64,PHN2ZyBpZD0iTGF5ZXJfMSIgZGF0YS1uYW1lPSJMYXllciAxIiB4bWxucz0iaHR0cDovL3d3dy53My5vcmcvMjAwMC9zdmciIHhtbG5zOnhsaW5rPSJodHRwOi8vd3d3LnczLm9yZy8xOTk5L3hsaW5rIiB2aWV3Qm94PSIwIDAgMTIxIDEyMSI+PGRlZnM+PHN0eWxlPi5jbHMtMXtmaWxsOnVybCgjbGluZWFyLWdyYWRpZW50KTt9LmNscy0yLC5jbHMtM3tmaWxsOiNkMWQxZDE7fS5jbHMtM3tzdHJva2U6I2I3YjdiNztzdHJva2UtbWl0ZXJsaW1pdDoxMDtzdHJva2Utd2lkdGg6MC4yNXB4O30uY2xzLTR7ZmlsbDojZjMwMDAwO30uY2xzLTV7ZmlsbDojZjIxNzY3O308L3N0eWxlPjxsaW5lYXJHcmFkaWVudCBpZD0ibGluZWFyLWdyYWRpZW50IiB4MT0iNjAuNSIgeTE9IjEyMC41IiB4Mj0iNjAuNSIgeTI9IjAuNSIgZ3JhZGllbnRVbml0cz0idXNlclNwYWNlT25Vc2UiPjxzdG9wIG9mZnNldD0iMCIgc3RvcC1jb2xvcj0iI2QxZDFkMSIvPjxzdG9wIG9mZnNldD0iMC4xIiBzdG9wLWNvbG9yPSIjY2VjZWNlIi8+PHN0b3Agb2Zmc2V0PSIwLjE5IiBzdG9wLWNvbG9yPSIjYzNjM2MzIi8+PHN0b3Agb2Zmc2V0PSIwLjI4IiBzdG9wLWNvbG9yPSIjYjFiMWIxIi8+PHN0b3Agb2Zmc2V0PSIwLjM2IiBzdG9wLWNvbG9yPSIjOTg5ODk4Ii8+PHN0b3Agb2Zmc2V0PSIwLjQ0IiBzdG9wLWNvbG9yPSIjNzg3ODc4Ii8+PHN0b3Agb2Zmc2V0PSIwLjQ2IiBzdG9wLWNvbG9yPSIjNmI2YjZiIi8+PHN0b3Agb2Zmc2V0PSIwLjU0IiBzdG9wLWNvbG9yPSIjNmI2YjZiIi8+PHN0b3Agb2Zmc2V0PSIwLjU2IiBzdG9wLWNvbG9yPSIjNzY3Njc2Ii8+PHN0b3Agb2Zmc2V0PSIwLjY0IiBzdG9wLWNvbG9yPSIjOTc5Nzk3Ii8+PHN0b3Agb2Zmc2V0PSIwLjcyIiBzdG9wLWNvbG9yPSIjYjBiMGIwIi8+PHN0b3Agb2Zmc2V0PSIwLjgxIiBzdG9wLWNvbG9yPSIjYzNjM2MzIi8+PHN0b3Agb2Zmc2V0PSIwLjkiIHN0b3AtY29sb3I9IiNjZGNkY2QiLz48c3RvcCBvZmZzZXQ9IjEiIHN0b3AtY29sb3I9IiNkMWQxZDEiLz48L2xpbmVhckdyYWRpZW50PjwvZGVmcz48Y2lyY2xlIGNsYXNzPSJjbHMtMSIgY3g9IjYwLjUiIGN5PSI2MC41IiByPSI2MCIvPjxwYXRoIGNsYXNzPSJjbHMtMiIgZD0iTTYwLjUsMUE1OS41LDU5LjUsMCwxLDEsMSw2MC41LDU5LjU3LDU5LjU3LDAsMCwxLDYwLjUsMW0wLTFBNjAuNSw2MC41LDAsMSwwLDEyMSw2MC41LDYwLjUsNjAuNSwwLDAsMCw2MC41LDBaIi8+PHJlY3QgY2xhc3M9ImNscy0zIiB4PSIwLjUiIHk9IjUxLjUiIHdpZHRoPSIxMjAiIGhlaWdodD0iMTgiIHJ4PSIzLjA0Ii8+PHJlY3QgY2xhc3M9ImNscy00IiB4PSI1Ljc1IiB5PSI1OC43NSIgd2lkdGg9IjE2IiBoZWlnaHQ9IjMiLz48cGF0aCBjbGFzcz0iY2xzLTUiIGQ9Ik0yMS4yNSw1OS4yNXYyaC0xNXYtMmgxNW0xLTFoLTE3djRoMTd2LTRaIi8+PC9zdmc+\"},\"handleOffset\":[0,0],\"handleOrientation\":180,\"handlePosition\":[0,0,1,1],\"handleSize\":{\"height\":0.5,\"width\":0.5},\"labelRadius\":0.36,\"position\":[0,0,1,1],\"states\":[{\"Label\":{\"color\":[0,0,0,1],\"icon\":{\"size\":[0,0],\"src\":[],\"srcOrientation\":\"Right\"},\"iconOffset\":0,\"iconPlacement\":\"left\",\"opacity\":1,\"position\":[0.7345552884615385,0.6796274038461538],\"show\":true,\"text\":{\"content\":\"Off\",\"font\":\"Helvetica\"}},\"Value\":0},{\"Label\":{\"color\":[0,0,0,1],\"icon\":{\"size\":[0,0],\"src\":[],\"srcOrientation\":\"Right\"},\"iconOffset\":0,\"iconPlacement\":\"left\",\"opacity\":1,\"position\":[0.7191706730769231,0.19501201923076922],\"show\":true,\"text\":{\"content\":\"1\",\"font\":\"Helvetica\"}},\"Value\":10000},{\"Label\":{\"color\":[0,0,0,1],\"icon\":{\"size\":[0,0],\"src\":[],\"srcOrientation\":\"Right\"},\"iconOffset\":0,\"iconPlacement\":\"left\",\"opacity\":1,\"position\":[0.7191706730769231,0.19501201923076922],\"show\":true,\"text\":{\"content\":\"2\",\"font\":\"Helvetica\"}},\"Value\":20000},{\"Label\":{\"color\":[0,0,0,1],\"icon\":{\"size\":[0,0],\"src\":[],\"srcOrientation\":\"Right\"},\"iconOffset\":0,\"iconPlacement\":\"left\",\"opacity\":1,\"position\":[0.7191706730769231,0.19501201923076922],\"show\":true,\"text\":{\"content\":\"3\",\"font\":\"Helvetica\"}},\"Value\":30000},{\"Label\":{\"color\":[0,0,0,1],\"icon\":{\"size\":[0,0],\"src\":[],\"srcOrientation\":\"Right\"},\"iconOffset\":0,\"iconPlacement\":\"left\",\"opacity\":1,\"position\":[0.7191706730769231,0.19501201923076922],\"show\":true,\"text\":{\"content\":\"4\",\"font\":\"Helvetica\"}},\"Value\":40000},{\"Label\":{\"color\":[0,0,0,1],\"icon\":{\"size\":[0,0],\"src\":[],\"srcOrientation\":\"Right\"},\"iconOffset\":0,\"iconPlacement\":\"left\",\"opacity\":1,\"position\":[0.7191706730769231,0.19501201923076922],\"show\":true,\"text\":{\"content\":\"5\",\"font\":\"Helvetica\"}},\"Value\":50000},{\"Label\":{\"color\":[0,0,0,1],\"icon\":{\"size\":[0,0],\"src\":[],\"srcOrientation\":\"Right\"},\"iconOffset\":0,\"iconPlacement\":\"left\",\"opacity\":1,\"position\":[0.7191706730769231,0.19501201923076922],\"show\":true,\"text\":{\"content\":\"6\",\"font\":\"Helvetica\"}},\"Value\":60000},{\"Label\":{\"color\":[0,0,0,1],\"icon\":{\"size\":[0,0],\"src\":[],\"srcOrientation\":\"Right\"},\"iconOffset\":0,\"iconPlacement\":\"left\",\"opacity\":1,\"position\":[0.7191706730769231,0.19501201923076922],\"show\":true,\"text\":{\"content\":\"6.5\",\"font\":\"Helvetica\"}},\"Value\":65000},{\"Label\":{\"color\":[0,0,0,1],\"icon\":{\"size\":[0,0],\"src\":[],\"srcOrientation\":\"Right\"},\"iconOffset\":0,\"iconPlacement\":\"left\",\"opacity\":1,\"position\":[0.7191706730769231,0.19501201923076922],\"show\":true,\"text\":{\"content\":\"7\",\"font\":\"Helvetica\"}},\"Value\":70000},{\"Label\":{\"color\":[0,0,0,1],\"icon\":{\"size\":[0,0],\"src\":[],\"srcOrientation\":\"Right\"},\"iconOffset\":0,\"iconPlacement\":\"left\",\"opacity\":1,\"position\":[0.7191706730769231,0.19501201923076922],\"show\":true,\"text\":{\"content\":\"7.5\",\"font\":\"Helvetica\"}},\"Value\":75000},{\"Label\":{\"color\":[0,0,0,1],\"icon\":{\"size\":[0,0],\"src\":[],\"srcOrientation\":\"Right\"},\"iconOffset\":0,\"iconPlacement\":\"left\",\"opacity\":1,\"position\":[0.7191706730769231,0.19501201923076922],\"show\":true,\"text\":{\"content\":\"8\",\"font\":\"Helvetica\"}},\"Value\":80000},{\"Label\":{\"color\":[0,0,0,1],\"icon\":{\"size\":[0,0],\"src\":[],\"srcOrientation\":\"Right\"},\"iconOffset\":0,\"iconPlacement\":\"left\",\"opacity\":1,\"position\":[0.7191706730769231,0.19501201923076922],\"show\":true,\"text\":{\"content\":\"8.5\",\"font\":\"Helvetica\"}},\"Value\":85000},{\"Label\":{\"color\":[0,0,0,1],\"icon\":{\"size\":[0,0],\"src\":[],\"srcOrientation\":\"Right\"},\"iconOffset\":0,\"iconPlacement\":\"left\",\"opacity\":1,\"position\":[0.7191706730769231,0.19501201923076922],\"show\":true,\"text\":{\"content\":\"9\",\"font\":\"Helvetica\"}},\"Value\":90000},{\"Label\":{\"color\":[0,0,0,1],\"icon\":{\"size\":[0,0],\"src\":[],\"srcOrientation\":\"Right\"},\"iconOffset\":0,\"iconPlacement\":\"left\",\"opacity\":1,\"position\":[0.7191706730769231,0.19501201923076922],\"show\":true,\"text\":{\"content\":\"9.5\",\"font\":\"Helvetica\"}},\"Value\":95000},{\"Label\":{\"color\":[0,0,0,1],\"icon\":{\"size\":[0,0],\"src\":[],\"srcOrientation\":\"Right\"},\"iconOffset\":0,\"iconPlacement\":\"left\",\"opacity\":1,\"position\":[0.7191706730769231,0.19501201923076922],\"show\":true,\"text\":{\"content\":\"10\",\"font\":\"Helvetica\"}},\"Value\":100000},{\"Label\":{\"color\":[0,0,0,1],\"icon\":{\"size\":[0,0],\"src\":[],\"srcOrientation\":\"Right\"},\"iconOffset\":0,\"iconPlacement\":\"left\",\"opacity\":1,\"position\":[0.7191706730769231,0.19501201923076922],\"show\":true,\"text\":{\"content\":\"10.5\",\"font\":\"Helvetica\"}},\"Value\":105000},{\"Label\":{\"color\":[0,0,0,1],\"icon\":{\"size\":[0,0],\"src\":[],\"srcOrientation\":\"Right\"},\"iconOffset\":0,\"iconPlacement\":\"left\",\"opacity\":1,\"position\":[0.7191706730769231,0.19501201923076922],\"show\":true,\"text\":{\"content\":\"11\",\"font\":\"Helvetica\"}},\"Value\":110000},{\"Label\":{\"color\":[0,0,0,1],\"icon\":{\"size\":[0,0],\"src\":[],\"srcOrientation\":\"Right\"},\"iconOffset\":0,\"iconPlacement\":\"left\",\"opacity\":1,\"position\":[0.7191706730769231,0.19501201923076922],\"show\":true,\"text\":{\"content\":\"11.5\",\"font\":\"Helvetica\"}},\"Value\":115000},{\"Label\":{\"color\":[0,0,0,1],\"icon\":{\"size\":[0,0],\"src\":[],\"srcOrientation\":\"Right\"},\"iconOffset\":0,\"iconPlacement\":\"left\",\"opacity\":1,\"position\":[0.7191706730769231,0.19501201923076922],\"show\":true,\"text\":{\"content\":\"12\",\"font\":\"Helvetica\"}},\"Value\":120000}],\"tickRadius\":0.32}},{\"name\":\"BackgroundImageComponent\",\"settings\":{\"image\":{\"size\":[155,150],\"src\":\"data:image\\/svg+xml;base64,PD94bWwgdmVyc2lvbj0iMS4wIiBlbmNvZGluZz0idXRmLTgiPz4NCjwhLS0gR2VuZXJhdG9yOiBBZG9iZSBJbGx1c3RyYXRvciAyNS4wLjAsIFNWRyBFeHBvcnQgUGx1Zy1JbiAuIFNWRyBWZXJzaW9uOiA2LjAwIEJ1aWxkIDApICAtLT4NCjxzdmcgdmVyc2lvbj0iMS4xIg0KCSBpZD0iTGF5ZXJfMl8xXyIgeG1sbnM6Y2M9Imh0dHA6Ly9jcmVhdGl2ZWNvbW1vbnMub3JnL25zIyIgeG1sbnM6ZGM9Imh0dHA6Ly9wdXJsLm9yZy9kYy9lbGVtZW50cy8xLjEvIiB4bWxuczppbmtzY2FwZT0iaHR0cDovL3d3dy5pbmtzY2FwZS5vcmcv ...(+4184 chars)\",\"srcOrientation\":\"Right\"},\"position\":[0,0,1,1],\"scaleMode\":\"0\"}},{\"name\":\"ForegroundImageComponent\",\"settings\":{\"image\":{\"size\":[0,0],\"src\":\"default\",\"srcOrientation\":[]},\"isForeground\":1,\"position\":[0,0,1,1],\"scaleMode\":\"0\"}}],\"settings\":{\"BindingType\":\"param\",\"backgroundColor\":[0,0,255,\"1\"],\"backgroundOffset\":1,\"fixedAspectRatio\":\"on\",\"image\":{\"size\":[150,150],\"src\":\"data:image\\/svg+xml;base64,PD94bWwgdmVyc2lvbj0iMS4wIiBlbmNvZGluZz0iVVRGLTgiIHN0YW5kYWxvbmU9Im5vIj8+CjwhLS0gR2VuZXJhdG9yOiBBZG9iZSBJbGx1c3RyYXRvciAxOS4yLjEsIFNWRyBFeHBvcnQgUGx1Zy1JbiAuIFNWRyBWZXJzaW9uOiA2LjAwIEJ1aWxkIDApICAtLT4KCjxzdmcKICAgeG1sbnM6ZGM9Imh0dHA6Ly9wdXJsLm9yZy9kYy9lbGVtZW50cy8xLjEvIgogICB4bWxuczpjYz0iaHR0cDovL2NyZWF0aXZlY29tbW9ucy5vcmcvbnMjIgogICB4bWxuczpyZGY9Imh0dHA6Ly93d3cudzMub3JnLzE5OTkvMDIvMjItcmRmLXN5bnRh ...(+9660 chars)\"},\"showBackgroundColor\":false,\"variant\":\"rotarySwitch\",\"version\":\"R2023a\"},\"type\":\"RotarySwitch\"}"
  Stepper Frequency : Constant  Value=80000
  Subsystem : Subsystem
  Subsystem1 : Subsystem
  Subsystem2 : Subsystem
  Sum : Sum  Inputs=|++
  Time Factor : CustomTuningWebBlock  LabelPosition=Hide  ShowInitialText=on  Configuration="{\"components\":[{\"name\":\"RotarySwitchComponent\",\"settings\":{\"arcAngle\":300,\"arcAngleOffset\":120,\"handle\":{\"size\":[150,150],\"src\":\"data:image\\/svg+xml;base64,PHN2ZyBpZD0iTGF5ZXJfMSIgZGF0YS1uYW1lPSJMYXllciAxIiB4bWxucz0iaHR0cDovL3d3dy53My5vcmcvMjAwMC9zdmciIHhtbG5zOnhsaW5rPSJodHRwOi8vd3d3LnczLm9yZy8xOTk5L3hsaW5rIiB2aWV3Qm94PSIwIDAgMTIxIDEyMSI+PGRlZnM+PHN0eWxlPi5jbHMtMXtmaWxsOnVybCgjbGluZWFyLWdyYWRpZW50KTt9LmNscy0yLC5jbHMtM3tmaWxsOiNkMWQxZDE7fS5jbHMtM3tzdHJva2U6I2I3YjdiNztzdHJva2UtbWl0ZXJsaW1pdDoxMDtzdHJva2Utd2lkdGg6MC4yNXB4O30uY2xzLTR7ZmlsbDojZjMwMDAwO30uY2xzLTV7ZmlsbDojZjIxNzY3O308L3N0eWxlPjxsaW5lYXJHcmFkaWVudCBpZD0ibGluZWFyLWdyYWRpZW50IiB4MT0iNjAuNSIgeTE9IjEyMC41IiB4Mj0iNjAuNSIgeTI9IjAuNSIgZ3JhZGllbnRVbml0cz0idXNlclNwYWNlT25Vc2UiPjxzdG9wIG9mZnNldD0iMCIgc3RvcC1jb2xvcj0iI2QxZDFkMSIvPjxzdG9wIG9mZnNldD0iMC4xIiBzdG9wLWNvbG9yPSIjY2VjZWNlIi8+PHN0b3Agb2Zmc2V0PSIwLjE5IiBzdG9wLWNvbG9yPSIjYzNjM2MzIi8+PHN0b3Agb2Zmc2V0PSIwLjI4IiBzdG9wLWNvbG9yPSIjYjFiMWIxIi8+PHN0b3Agb2Zmc2V0PSIwLjM2IiBzdG9wLWNvbG9yPSIjOTg5ODk4Ii8+PHN0b3Agb2Zmc2V0PSIwLjQ0IiBzdG9wLWNvbG9yPSIjNzg3ODc4Ii8+PHN0b3Agb2Zmc2V0PSIwLjQ2IiBzdG9wLWNvbG9yPSIjNmI2YjZiIi8+PHN0b3Agb2Zmc2V0PSIwLjU0IiBzdG9wLWNvbG9yPSIjNmI2YjZiIi8+PHN0b3Agb2Zmc2V0PSIwLjU2IiBzdG9wLWNvbG9yPSIjNzY3Njc2Ii8+PHN0b3Agb2Zmc2V0PSIwLjY0IiBzdG9wLWNvbG9yPSIjOTc5Nzk3Ii8+PHN0b3Agb2Zmc2V0PSIwLjcyIiBzdG9wLWNvbG9yPSIjYjBiMGIwIi8+PHN0b3Agb2Zmc2V0PSIwLjgxIiBzdG9wLWNvbG9yPSIjYzNjM2MzIi8+PHN0b3Agb2Zmc2V0PSIwLjkiIHN0b3AtY29sb3I9IiNjZGNkY2QiLz48c3RvcCBvZmZzZXQ9IjEiIHN0b3AtY29sb3I9IiNkMWQxZDEiLz48L2xpbmVhckdyYWRpZW50PjwvZGVmcz48Y2lyY2xlIGNsYXNzPSJjbHMtMSIgY3g9IjYwLjUiIGN5PSI2MC41IiByPSI2MCIvPjxwYXRoIGNsYXNzPSJjbHMtMiIgZD0iTTYwLjUsMUE1OS41LDU5LjUsMCwxLDEsMSw2MC41LDU5LjU3LDU5LjU3LDAsMCwxLDYwLjUsMW0wLTFBNjAuNSw2MC41LDAsMSwwLDEyMSw2MC41LDYwLjUsNjAuNSwwLDAsMCw2MC41LDBaIi8+PHJlY3QgY2xhc3M9ImNscy0zIiB4PSIwLjUiIHk9IjUxLjUiIHdpZHRoPSIxMjAiIGhlaWdodD0iMTgiIHJ4PSIzLjA0Ii8+PHJlY3QgY2xhc3M9ImNscy00IiB4PSI1Ljc1IiB5PSI1OC43NSIgd2lkdGg9IjE2IiBoZWlnaHQ9IjMiLz48cGF0aCBjbGFzcz0iY2xzLTUiIGQ9Ik0yMS4yNSw1OS4yNXYyaC0xNXYtMmgxNW0xLTFoLTE3djRoMTd2LTRaIi8+PC9zdmc+\"},\"handleOffset\":[0,0],\"handleOrientation\":180,\"handlePosition\":[0,0,1,1],\"handleSize\":{\"height\":0.5,\"width\":0.5},\"labelRadius\":0.36,\"position\":[0,0,1,1],\"states\":[{\"Label\":{\"color\":[0,0,0,1],\"icon\":{\"size\":[0,0],\"src\":[],\"srcOrientation\":\"Right\"},\"iconOffset\":0,\"iconPlacement\":\"left\",\"opacity\":1,\"position\":[0.7345552884615385,0.6796274038461538],\"show\":true,\"text\":{\"content\":\"0\",\"font\":\"Helvetica\"}},\"Value\":0},{\"Label\":{\"color\":[0,0,0,1],\"icon\":{\"size\":[0,0],\"src\":[],\"srcOrientation\":\"Right\"},\"iconOffset\":0,\"iconPlacement\":\"left\",\"opacity\":1,\"position\":[0.7191706730769231,0.19501201923076922],\"show\":true,\"text\":{\"content\":\"1\",\"font\":\"Helvetica\"}},\"Value\":1},{\"Label\":{\"color\":[0,0,0,1],\"icon\":{\"size\":[0,0],\"src\":[],\"srcOrientation\":\"Right\"},\"iconOffset\":0,\"iconPlacement\":\"left\",\"opacity\":1,\"position\":[0.7191706730769231,0.19501201923076922],\"show\":true,\"text\":{\"content\":\"10\",\"font\":\"Helvetica\"}},\"Value\":2},{\"Label\":{\"color\":[0,0,0,1],\"icon\":{\"size\":[0,0],\"src\":[],\"srcOrientation\":\"Right\"},\"iconOffset\":0,\"iconPlacement\":\"left\",\"opacity\":1,\"position\":[0.7191706730769231,0.19501201923076922],\"show\":true,\"text\":{\"content\":\"50\",\"font\":\"Helvetica\"}},\"Value\":3},{\"Label\":{\"color\":[0,0,0,1],\"icon\":{\"size\":[0,0],\"src\":[],\"srcOrientation\":\"Right\"},\"iconOffset\":0,\"iconPlacement\":\"left\",\"opacity\":1,\"position\":[0.7191706730769231,0.19501201923076922],\"show\":true,\"text\":{\"content\":\"100\",\"font\":\"Helvetica\"}},\"Value\":4},{\"Label\":{\"color\":[0,0,0,1],\"icon\":{\"size\":[0,0],\"src\":[],\"srcOrientation\":\"Right\"},\"iconOffset\":0,\"iconPlacement\":\"left\",\"opacity\":1,\"position\":[0.7191706730769231,0.19501201923076922],\"show\":true,\"text\":{\"content\":\"500\",\"font\":\"Helvetica\"}},\"Value\":5},{\"Label\":{\"color\":[0,0,0,1],\"icon\":{\"size\":[0,0],\"src\":[],\"srcOrientation\":\"Right\"},\"iconOffset\":0,\"iconPlacement\":\"left\",\"opacity\":1,\"position\":[0.7191706730769231,0.19501201923076922],\"show\":true,\"text\":{\"content\":\"1000\",\"font\":\"Helvetica\"}},\"Value\":6},{\"Label\":{\"color\":[0,0,0,1],\"icon\":{\"size\":[0,0],\"src\":[],\"srcOrientation\":\"Right\"},\"iconOffset\":0,\"iconPlacement\":\"left\",\"opacity\":1,\"position\":[0.7191706730769231,0.19501201923076922],\"show\":true,\"text\":{\"content\":\"5000\",\"font\":\"Helvetica\"}},\"Value\":7},{\"Label\":{\"color\":[0,0,0,1],\"icon\":{\"size\":[0,0],\"src\":[],\"srcOrientation\":\"Right\"},\"iconOffset\":0,\"iconPlacement\":\"left\",\"opacity\":1,\"position\":[0.7191706730769231,0.19501201923076922],\"show\":true,\"text\":{\"content\":\"10000\",\"font\":\"Helvetica\"}},\"Value\":8},{\"Label\":{\"color\":[0,0,0,1],\"icon\":{\"size\":[0,0],\"src\":[],\"srcOrientation\":\"Right\"},\"iconOffset\":0,\"iconPlacement\":\"left\",\"opacity\":1,\"position\":[0.7191706730769231,0.19501201923076922],\"show\":true,\"text\":{\"content\":\"20000\",\"font\":\"Helvetica\"}},\"Value\":9},{\"Label\":{\"color\":[0,0,0,1],\"icon\":{\"size\":[0,0],\"src\":[],\"srcOrientation\":\"Right\"},\"iconOffset\":0,\"iconPlacement\":\"left\",\"opacity\":1,\"position\":[0.7191706730769231,0.19501201923076922],\"show\":true,\"text\":{\"content\":\"50000\",\"font\":\"Helvetica\"}},\"Value\":10},{\"Label\":{\"color\":[0,0,0,1],\"icon\":{\"size\":[0,0],\"src\":[],\"srcOrientation\":\"Right\"},\"iconOffset\":0,\"iconPlacement\":\"left\",\"opacity\":1,\"position\":[0.7191706730769231,0.19501201923076922],\"show\":true,\"text\":{\"content\":\"75000\",\"font\":\"Helvetica\"}},\"Value\":11},{\"Label\":{\"color\":[0,0,0,1],\"icon\":{\"size\":[0,0],\"src\":[],\"srcOrientation\":\"Right\"},\"iconOffset\":0,\"iconPlacement\":\"left\",\"opacity\":1,\"position\":[0.7191706730769231,0.19501201923076922],\"show\":true,\"text\":{\"content\":\"100000\",\"font\":\"Helvetica\"}},\"Value\":12}],\"tickRadius\":0.32}},{\"name\":\"BackgroundImageComponent\",\"settings\":{\"image\":{\"size\":[155,150],\"src\":\"data:image\\/svg+xml;base64,PD94bWwgdmVyc2lvbj0iMS4wIiBlbmNvZGluZz0idXRmLTgiPz4NCjwhLS0gR2VuZXJhdG9yOiBBZG9iZSBJbGx1c3RyYXRvciAyNS4wLjAsIFNWRyBFeHBvcnQgUGx1Zy1JbiAuIFNWRyBWZXJzaW9uOiA2LjAwIEJ1aWxkIDApICAtLT4NCjxzdmcgdmVyc2lvbj0iMS4xIg0KCSBpZD0iTGF5ZXJfMl8xXyIgeG1sbnM6Y2M9Imh0dHA6Ly9jcmVhdGl2ZWNvbW1vbnMub3JnL25zIyIgeG1sbnM6ZGM9Imh0dHA6Ly9wdXJsLm9yZy9kYy9lbGVtZW50cy8xLjEvIiB4bWxuczppbmtzY2FwZT0iaHR0cDovL3d3dy5pbmtzY2FwZS5vcmcv ...(+4184 chars)\",\"srcOrientation\":\"Right\"},\"position\":[0,0,1,1],\"scaleMode\":\"0\"}},{\"name\":\"ForegroundImageComponent\",\"settings\":{\"image\":{\"size\":[0,0],\"src\":\"default\",\"srcOrientation\":[]},\"isForeground\":1,\"position\":[0,0,1,1],\"scaleMode\":\"0\"}}],\"settings\":{\"BindingType\":\"param\",\"backgroundColor\":[0,0,255,\"1\"],\"backgroundOffset\":1,\"fixedAspectRatio\":\"on\",\"image\":{\"size\":[150,150],\"src\":\"data:image\\/svg+xml;base64,PD94bWwgdmVyc2lvbj0iMS4wIiBlbmNvZGluZz0iVVRGLTgiIHN0YW5kYWxvbmU9Im5vIj8+CjwhLS0gR2VuZXJhdG9yOiBBZG9iZSBJbGx1c3RyYXRvciAxOS4yLjEsIFNWRyBFeHBvcnQgUGx1Zy1JbiAuIFNWRyBWZXJzaW9uOiA2LjAwIEJ1aWxkIDApICAtLT4KCjxzdmcKICAgeG1sbnM6ZGM9Imh0dHA6Ly9wdXJsLm9yZy9kYy9lbGVtZW50cy8xLjEvIgogICB4bWxuczpjYz0iaHR0cDovL2NyZWF0aXZlY29tbW9ucy5vcmcvbnMjIgogICB4bWxuczpyZGY9Imh0dHA6Ly93d3cudzMub3JnLzE5OTkvMDIvMjItcmRmLXN5bnRh ...(+9660 chars)\"},\"showBackgroundColor\":false,\"variant\":\"rotarySwitch\",\"version\":\"R2023a\"},\"type\":\"RotarySwitch\"}"
  Time Factor2 : CustomTuningWebBlock  LabelPosition=Hide  ShowInitialText=on  Configuration="{\"components\":[{\"name\":\"RotarySwitchComponent\",\"settings\":{\"arcAngle\":300,\"arcAngleOffset\":120,\"handle\":{\"size\":[150,150],\"src\":\"data:image\\/svg+xml;base64,PHN2ZyBpZD0iTGF5ZXJfMSIgZGF0YS1uYW1lPSJMYXllciAxIiB4bWxucz0iaHR0cDovL3d3dy53My5vcmcvMjAwMC9zdmciIHhtbG5zOnhsaW5rPSJodHRwOi8vd3d3LnczLm9yZy8xOTk5L3hsaW5rIiB2aWV3Qm94PSIwIDAgMTIxIDEyMSI+PGRlZnM+PHN0eWxlPi5jbHMtMXtmaWxsOnVybCgjbGluZWFyLWdyYWRpZW50KTt9LmNscy0yLC5jbHMtM3tmaWxsOiNkMWQxZDE7fS5jbHMtM3tzdHJva2U6I2I3YjdiNztzdHJva2UtbWl0ZXJsaW1pdDoxMDtzdHJva2Utd2lkdGg6MC4yNXB4O30uY2xzLTR7ZmlsbDojZjMwMDAwO30uY2xzLTV7ZmlsbDojZjIxNzY3O308L3N0eWxlPjxsaW5lYXJHcmFkaWVudCBpZD0ibGluZWFyLWdyYWRpZW50IiB4MT0iNjAuNSIgeTE9IjEyMC41IiB4Mj0iNjAuNSIgeTI9IjAuNSIgZ3JhZGllbnRVbml0cz0idXNlclNwYWNlT25Vc2UiPjxzdG9wIG9mZnNldD0iMCIgc3RvcC1jb2xvcj0iI2QxZDFkMSIvPjxzdG9wIG9mZnNldD0iMC4xIiBzdG9wLWNvbG9yPSIjY2VjZWNlIi8+PHN0b3Agb2Zmc2V0PSIwLjE5IiBzdG9wLWNvbG9yPSIjYzNjM2MzIi8+PHN0b3Agb2Zmc2V0PSIwLjI4IiBzdG9wLWNvbG9yPSIjYjFiMWIxIi8+PHN0b3Agb2Zmc2V0PSIwLjM2IiBzdG9wLWNvbG9yPSIjOTg5ODk4Ii8+PHN0b3Agb2Zmc2V0PSIwLjQ0IiBzdG9wLWNvbG9yPSIjNzg3ODc4Ii8+PHN0b3Agb2Zmc2V0PSIwLjQ2IiBzdG9wLWNvbG9yPSIjNmI2YjZiIi8+PHN0b3Agb2Zmc2V0PSIwLjU0IiBzdG9wLWNvbG9yPSIjNmI2YjZiIi8+PHN0b3Agb2Zmc2V0PSIwLjU2IiBzdG9wLWNvbG9yPSIjNzY3Njc2Ii8+PHN0b3Agb2Zmc2V0PSIwLjY0IiBzdG9wLWNvbG9yPSIjOTc5Nzk3Ii8+PHN0b3Agb2Zmc2V0PSIwLjcyIiBzdG9wLWNvbG9yPSIjYjBiMGIwIi8+PHN0b3Agb2Zmc2V0PSIwLjgxIiBzdG9wLWNvbG9yPSIjYzNjM2MzIi8+PHN0b3Agb2Zmc2V0PSIwLjkiIHN0b3AtY29sb3I9IiNjZGNkY2QiLz48c3RvcCBvZmZzZXQ9IjEiIHN0b3AtY29sb3I9IiNkMWQxZDEiLz48L2xpbmVhckdyYWRpZW50PjwvZGVmcz48Y2lyY2xlIGNsYXNzPSJjbHMtMSIgY3g9IjYwLjUiIGN5PSI2MC41IiByPSI2MCIvPjxwYXRoIGNsYXNzPSJjbHMtMiIgZD0iTTYwLjUsMUE1OS41LDU5LjUsMCwxLDEsMSw2MC41LDU5LjU3LDU5LjU3LDAsMCwxLDYwLjUsMW0wLTFBNjAuNSw2MC41LDAsMSwwLDEyMSw2MC41LDYwLjUsNjAuNSwwLDAsMCw2MC41LDBaIi8+PHJlY3QgY2xhc3M9ImNscy0zIiB4PSIwLjUiIHk9IjUxLjUiIHdpZHRoPSIxMjAiIGhlaWdodD0iMTgiIHJ4PSIzLjA0Ii8+PHJlY3QgY2xhc3M9ImNscy00IiB4PSI1Ljc1IiB5PSI1OC43NSIgd2lkdGg9IjE2IiBoZWlnaHQ9IjMiLz48cGF0aCBjbGFzcz0iY2xzLTUiIGQ9Ik0yMS4yNSw1OS4yNXYyaC0xNXYtMmgxNW0xLTFoLTE3djRoMTd2LTRaIi8+PC9zdmc+\"},\"handleOffset\":[0,0],\"handleOrientation\":180,\"handlePosition\":[0,0,1,1],\"handleSize\":{\"height\":0.5,\"width\":0.5},\"labelRadius\":0.36,\"position\":[0,0,1,1],\"states\":[{\"Label\":{\"color\":[0,0,0,1],\"icon\":{\"size\":[0,0],\"src\":[],\"srcOrientation\":\"Right\"},\"iconOffset\":0,\"iconPlacement\":\"left\",\"opacity\":1,\"position\":[0.7345552884615385,0.6796274038461538],\"show\":true,\"text\":{\"content\":\"0\",\"font\":\"Helvetica\"}},\"Value\":0},{\"Label\":{\"color\":[0,0,0,1],\"icon\":{\"size\":[0,0],\"src\":[],\"srcOrientation\":\"Right\"},\"iconOffset\":0,\"iconPlacement\":\"left\",\"opacity\":1,\"position\":[0.7191706730769231,0.19501201923076922],\"show\":true,\"text\":{\"content\":\"1\",\"font\":\"Helvetica\"}},\"Value\":1},{\"Label\":{\"color\":[0,0,0,1],\"icon\":{\"size\":[0,0],\"src\":[],\"srcOrientation\":\"Right\"},\"iconOffset\":0,\"iconPlacement\":\"left\",\"opacity\":1,\"position\":[0.7191706730769231,0.19501201923076922],\"show\":true,\"text\":{\"content\":\"10\",\"font\":\"Helvetica\"}},\"Value\":2},{\"Label\":{\"color\":[0,0,0,1],\"icon\":{\"size\":[0,0],\"src\":[],\"srcOrientation\":\"Right\"},\"iconOffset\":0,\"iconPlacement\":\"left\",\"opacity\":1,\"position\":[0.7191706730769231,0.19501201923076922],\"show\":true,\"text\":{\"content\":\"50\",\"font\":\"Helvetica\"}},\"Value\":3},{\"Label\":{\"color\":[0,0,0,1],\"icon\":{\"size\":[0,0],\"src\":[],\"srcOrientation\":\"Right\"},\"iconOffset\":0,\"iconPlacement\":\"left\",\"opacity\":1,\"position\":[0.7191706730769231,0.19501201923076922],\"show\":true,\"text\":{\"content\":\"100\",\"font\":\"Helvetica\"}},\"Value\":4},{\"Label\":{\"color\":[0,0,0,1],\"icon\":{\"size\":[0,0],\"src\":[],\"srcOrientation\":\"Right\"},\"iconOffset\":0,\"iconPlacement\":\"left\",\"opacity\":1,\"position\":[0.7191706730769231,0.19501201923076922],\"show\":true,\"text\":{\"content\":\"500\",\"font\":\"Helvetica\"}},\"Value\":5},{\"Label\":{\"color\":[0,0,0,1],\"icon\":{\"size\":[0,0],\"src\":[],\"srcOrientation\":\"Right\"},\"iconOffset\":0,\"iconPlacement\":\"left\",\"opacity\":1,\"position\":[0.7191706730769231,0.19501201923076922],\"show\":true,\"text\":{\"content\":\"1000\",\"font\":\"Helvetica\"}},\"Value\":6},{\"Label\":{\"color\":[0,0,0,1],\"icon\":{\"size\":[0,0],\"src\":[],\"srcOrientation\":\"Right\"},\"iconOffset\":0,\"iconPlacement\":\"left\",\"opacity\":1,\"position\":[0.7191706730769231,0.19501201923076922],\"show\":true,\"text\":{\"content\":\"5000\",\"font\":\"Helvetica\"}},\"Value\":7},{\"Label\":{\"color\":[0,0,0,1],\"icon\":{\"size\":[0,0],\"src\":[],\"srcOrientation\":\"Right\"},\"iconOffset\":0,\"iconPlacement\":\"left\",\"opacity\":1,\"position\":[0.7191706730769231,0.19501201923076922],\"show\":true,\"text\":{\"content\":\"10000\",\"font\":\"Helvetica\"}},\"Value\":8},{\"Label\":{\"color\":[0,0,0,1],\"icon\":{\"size\":[0,0],\"src\":[],\"srcOrientation\":\"Right\"},\"iconOffset\":0,\"iconPlacement\":\"left\",\"opacity\":1,\"position\":[0.7191706730769231,0.19501201923076922],\"show\":true,\"text\":{\"content\":\"20000\",\"font\":\"Helvetica\"}},\"Value\":9},{\"Label\":{\"color\":[0,0,0,1],\"icon\":{\"size\":[0,0],\"src\":[],\"srcOrientation\":\"Right\"},\"iconOffset\":0,\"iconPlacement\":\"left\",\"opacity\":1,\"position\":[0.7191706730769231,0.19501201923076922],\"show\":true,\"text\":{\"content\":\"50000\",\"font\":\"Helvetica\"}},\"Value\":10},{\"Label\":{\"color\":[0,0,0,1],\"icon\":{\"size\":[0,0],\"src\":[],\"srcOrientation\":\"Right\"},\"iconOffset\":0,\"iconPlacement\":\"left\",\"opacity\":1,\"position\":[0.7191706730769231,0.19501201923076922],\"show\":true,\"text\":{\"content\":\"75000\",\"font\":\"Helvetica\"}},\"Value\":11},{\"Label\":{\"color\":[0,0,0,1],\"icon\":{\"size\":[0,0],\"src\":[],\"srcOrientation\":\"Right\"},\"iconOffset\":0,\"iconPlacement\":\"left\",\"opacity\":1,\"position\":[0.7191706730769231,0.19501201923076922],\"show\":true,\"text\":{\"content\":\"100000\",\"font\":\"Helvetica\"}},\"Value\":12}],\"tickRadius\":0.32}},{\"name\":\"BackgroundImageComponent\",\"settings\":{\"image\":{\"size\":[155,150],\"src\":\"data:image\\/svg+xml;base64,PD94bWwgdmVyc2lvbj0iMS4wIiBlbmNvZGluZz0idXRmLTgiPz4NCjwhLS0gR2VuZXJhdG9yOiBBZG9iZSBJbGx1c3RyYXRvciAyNS4wLjAsIFNWRyBFeHBvcnQgUGx1Zy1JbiAuIFNWRyBWZXJzaW9uOiA2LjAwIEJ1aWxkIDApICAtLT4NCjxzdmcgdmVyc2lvbj0iMS4xIg0KCSBpZD0iTGF5ZXJfMl8xXyIgeG1sbnM6Y2M9Imh0dHA6Ly9jcmVhdGl2ZWNvbW1vbnMub3JnL25zIyIgeG1sbnM6ZGM9Imh0dHA6Ly9wdXJsLm9yZy9kYy9lbGVtZW50cy8xLjEvIiB4bWxuczppbmtzY2FwZT0iaHR0cDovL3d3dy5pbmtzY2FwZS5vcmcv ...(+4184 chars)\",\"srcOrientation\":\"Right\"},\"position\":[0,0,1,1],\"scaleMode\":\"0\"}},{\"name\":\"ForegroundImageComponent\",\"settings\":{\"image\":{\"size\":[0,0],\"src\":\"default\",\"srcOrientation\":[]},\"isForeground\":1,\"position\":[0,0,1,1],\"scaleMode\":\"0\"}}],\"settings\":{\"BindingType\":\"param\",\"backgroundColor\":[0,0,255,\"1\"],\"backgroundOffset\":1,\"fixedAspectRatio\":\"on\",\"image\":{\"size\":[150,150],\"src\":\"data:image\\/svg+xml;base64,PD94bWwgdmVyc2lvbj0iMS4wIiBlbmNvZGluZz0iVVRGLTgiIHN0YW5kYWxvbmU9Im5vIj8+CjwhLS0gR2VuZXJhdG9yOiBBZG9iZSBJbGx1c3RyYXRvciAxOS4yLjEsIFNWRyBFeHBvcnQgUGx1Zy1JbiAuIFNWRyBWZXJzaW9uOiA2LjAwIEJ1aWxkIDApICAtLT4KCjxzdmcKICAgeG1sbnM6ZGM9Imh0dHA6Ly9wdXJsLm9yZy9kYy9lbGVtZW50cy8xLjEvIgogICB4bWxuczpjYz0iaHR0cDovL2NyZWF0aXZlY29tbW9ucy5vcmcvbnMjIgogICB4bWxuczpyZGY9Imh0dHA6Ly93d3cudzMub3JnLzE5OTkvMDIvMjItcmRmLXN5bnRh ...(+9660 chars)\"},\"showBackgroundColor\":false,\"variant\":\"rotarySwitch\",\"version\":\"R2023a\"},\"type\":\"RotarySwitch\"}"
  Toggle Switch : CustomTuningWebBlock  LabelPosition=Hide  ShowInitialText=on  Configuration="{\"components\":[{\"name\":\"CustomSwitchStateComponent\",\"settings\":{\"position\":[0,0,1,1],\"showAllLabels\":1,\"states\":[{\"HitRegion\":{\"position\":[0,0,1,0.5]},\"Image\":{\"position\":[0,0.24928571428571428,0.5014285714285714,1],\"size\":[0.5014285714285714,1],\"src\":\"data:image\\/svg+xml;base64,PHN2ZyB4bWxucz0iaHR0cDovL3d3dy53My5vcmcvMjAwMC9zdmciIHhtbG5zOnhsaW5rPSJodHRwOi8vd3d3LnczLm9yZy8xOTk5L3hsaW5rIiB2aWV3Qm94PSIwIDAgMzguMDQgMTUwIj48ZGVmcz48c3R5bGU+LmNscy0xe2ZpbGw6dXJsKCNyYWRpYWwtZ3JhZGllbnQpO30uY2xzLTJ7ZmlsbDp1cmwoI3JhZGlhbC1ncmFkaWVudC0yKTt9LmNscy0ze2ZpbGw6dXJsKCNXaGl0ZV9CbGFjayk7fS5jbHMtNHtmaWxsOnVybCgjcmFkaWFsLWdyYWRpZW50LTMpO30uY2xzLTV7ZmlsbDojNWI1YjViO30uY2xzLTZ7ZmlsbDp1cmwoI3Jh ...(+3628 chars)\",\"srcOrientation\":\"Right\"},\"Label\":{\"color\":[0.5019607843137255,0.5019607843137255,0.5019607843137255],\"icon\":{\"size\":[0,0],\"src\":[],\"srcOrientation\":\"Right\"},\"iconOffset\":0,\"iconPlacement\":\"left\",\"opacity\":1,\"position\":[0.08,0.5],\"show\":true,\"text\":{\"content\":\"On\",\"font\":\"Helvetica\"}},\"Value\":0},{\"HitRegion\":{\"position\":[0.5,0,1,0.5]},\"Image\":{\"position\":[0,0.24928571428571428,0.5014285714285714,1],\"size\":[0.5014285714285714,1],\"src\":\"data:image\\/svg+xml;base64,PHN2ZyB4bWxucz0iaHR0cDovL3d3dy53My5vcmcvMjAwMC9zdmciIHhtbG5zOnhsaW5rPSJodHRwOi8vd3d3LnczLm9yZy8xOTk5L3hsaW5rIiB2aWV3Qm94PSIwIDAgMzguMDQgMTUwIj48ZGVmcz48c3R5bGU+LmNscy0xe2ZpbGw6dXJsKCNyYWRpYWwtZ3JhZGllbnQpO30uY2xzLTJ7ZmlsbDp1cmwoI3JhZGlhbC1ncmFkaWVudC0yKTt9LmNscy0ze2ZpbGw6dXJsKCNXaGl0ZV9CbGFjayk7fS5jbHMtNHtmaWxsOnVybCgjcmFkaWFsLWdyYWRpZW50LTMpO30uY2xzLTV7ZmlsbDojNWI1YjViO30uY2xzLTZ7ZmlsbDp1cmwoI3Jh ...(+3556 chars)\",\"srcOrientation\":\"Right\"},\"Label\":{\"color\":[0.5019607843137255,0.5019607843137255,0.5019607843137255],\"icon\":{\"size\":[0,0],\"src\":[],\"srcOrientation\":\"Right\"},\"iconOffset\":0,\"iconPlacement\":\"left\",\"opacity\":1,\"position\":[0.92,0.5],\"show\":true,\"text\":{\"content\":\"Off\",\"font\":\"Helvetica\"}},\"Value\":1}]}},{\"name\":\"BackgroundImageComponent\",\"settings\":{\"image\":{\"size\":[70,135],\"src\":\"default\",\"srcOrientation\":\"Right\"},\"position\":[0,0,1,1],\"scaleMode\":\"0\"}},{\"name\":\"ForegroundImageComponent\",\"settings\":{\"image\":{\"size\":[0,0],\"src\":\"default\",\"srcOrientation\":[]},\"isForeground\":1,\"position\":[0,0,1,1],\"scaleMode\":\"0\"}}],\"settings\":{\"BindingType\":\"param\",\"backgroundColor\":[0,0,0],\"backgroundOffset\":0.14,\"fixedAspectRatio\":\"on\",\"foregroundColor\":[0,0,0],\"showBackgroundColor\":false,\"variant\":\"toggle\",\"version\":\"R2024b\"},\"type\":\"Switch\"}"
  rad/s : Gain  Gain=2*pi/8192
  wcs1_offset_volt : Constant  Value=0.425  OutDataTypeStr=single
  wcs2_offset_volt : Constant  Value=0.318  OutDataTypeStr=single
  Out1 : Outport
  wires:
  Host Serial Rx1/2 -> Display8/1  "wcs1_raw_volt"
  Host Serial Rx1/3 -> Display16/1  "wcs2_raw_volt"
  Host Serial Rx1/7 -> Display6/1  "loadcell"
  Host Serial Rx1/5 -> Display2/1  "wcs2"
  Host Serial Rx1/8 -> Display7/1  "rawAngle"
  rad/s/1 -> Data Type Conversion3/1, Display5/1
  Host Serial Rx1/6 -> Display4/1, rad/s/1  "pps"
  Host Serial Rx1/4 -> Display1/1  "wcs1"
  Host Serial Rx1/9 -> Display3/1  "pulses"
  wcs1_offset_volt/1 -> Subsystem/1(wcs1_offset_volt)  "wcs1_offset_volt"
  wcs2_offset_volt/1 -> Subsystem/2(wcs2_offset_volt)  "wcs2_offset_volt"
  DC torque_setpoint/1 -> Subsystem/3(DC torque_setpoint)  "DC torque_setpoint"
  DC Frequency/1 -> Subsystem/5(DC Frequency)  "DC Frequency"
  DIR/1 -> Subsystem/9(DIR)  "DIR"
  EN/1 -> Subsystem/10(EN)  "EN"
  Subsystem/1(wcs1_offset_volt_out) -> Host Serial Tx/1
  Subsystem/2(wcs2_offset_volt_out) -> Host Serial Tx/2
  Subsystem/3(DC torque_setpoint1) -> Host Serial Tx/3
  Subsystem/4(Stepper Config) -> Host Serial Tx/4
  Subsystem/5(Stepper Frequency1) -> Host Serial Tx/5
  Subsystem/6(DC PWM1) -> Host Serial Tx/6
  Subsystem/7(DC Frequency1) -> Host Serial Tx/7
  Ramp/1 -> Display/1, Scope/1
  Stepper Frequency/1 -> FREQUENCY/1  "Stepper Frequency"
  Constant/1 -> MATLAB Function/1(u)
  MATLAB Function/1(m0) -> Subsystem/6(M0)
  MATLAB Function/2(m1) -> Subsystem/7(M1)
  MATLAB Function/3(m2) -> Subsystem/8(M2)
  FREQUENCY/1 -> Subsystem/11(Stepper Frequency), Out1/1, Display11/1
  Fine Value/1 -> FREQUENCY/2
  Fine 2/1 -> FREQUENCY/3
  Subsystem1/1(Out1) -> FREQUENCY/4, Display9/1
  Subsystem2/1(Out1) -> FREQUENCY1/2, Display12/1
  FREQUENCY1/1 -> FREQUENCY/5
  Data Type Conversion3/1 -> Lowpass Filter/1
  DC PWM/1 -> Subsystem/4(DC PWM)  "DC PWM"
  Constant5/1 -> Lowpass Filter/2
  Lowpass Filter/1 -> Loss Detector/2(angular_velocity), FilterRAD4/1
  Constant1/1 -> Loss Detector/4(steps_per_rev)
  frequency/1 -> Loss Detector/1(frequency)
  Loss Detector/2(lost_steps) -> Display10/1
  Loss Detector/3(position_error) -> Display14/1
  Loss Detector/1(step_loss_detected) -> Display15/1
  Sum/1 -> Loss Detector/3(elapsed_time)
  Clock/1 -> Display13/1, Sum/2
  Constant2/1 -> Sum/1
